simulink library "lib_TCML"  (R2015a)
settings: Solver=ode45  StartTime=0.0  StopTime=10.0  RelTol=1e-3
libraries: simulink x5
(part 1 of 7)
settings Model: Creator=jlkratz  LastModifiedBy=jlkratz

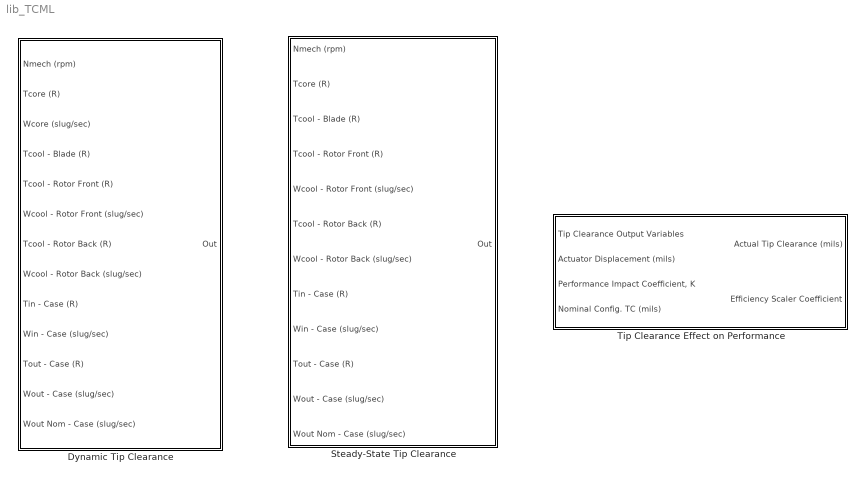
== system lib_TCML ==
  Dynamic Tip Clearance : Subsystem  mask(TCML - Dynamic Tip Clearance Library Block){m_Blade_M=0.0566, A_Blade_M=0.0174, Cp_TempDependence_Blade_M=on, Cp_Blade_M=4.5, TCp_Blade_Data_M=[0 10000], Cp_Blade_Data_M=[4.5 4.5], eta_Blade_M=0.5, T0_Blade_M=1800, dt_Blade_M=0.015, h_Const_Blade_M=off, h_Eqn_Blade_M=on, h_Data_Blade_M=off, h_Blade_M=0.03, hcoeff_Blade_M=0.03, Wdes_Blade_M=3, Tdes_Blade_M=1800, Wc_Blade_Data_M=[0 100], Tc_Blade_Data_M=[0 10], h_Blade_Data_M=[0.03 0.03; 0.03 0.03], L_Blade_M=0.125, rho_Blade_M=15.8975, alpha_TempDependence_Blade_M=on, alpha_Blade_M=0.000008, Talpha_Blade_Data_M=[0 10000], alpha_Blade_Data_M=[0.000008 0.000008], E_TempDependence_Blade_M=on, E_Blade_M=3974400000, TE_Blade_Data_M=[0 10000], E_Blade_Data_M=[3974400000 3974400000], W_Rotor_M=0.0833, n_Rotor_M=20, T0_Rotor_M=700*ones(1,20), dt_Rotor_M=0.06, rho_Rotor_M=15.8975, k_TempDependence_Rotor_M=on, k_Rotor_M=0.0015, Tk_Rotor_Data_M=[0 10000], k_Rotor_Data_M=[0.0015 0.0015], Cp_TempDependence_Rotor_M=on, Cp_Rotor_M=4.5, TCp_Rotor_Data_M=[0 10000], Cp_Rotor_Data_M=[4.5 4.5], h_Const_Rotor_Front_M=off, h_Eqn_Rotor_Front_M=on, h_Data_Rotor_Front_M=off, h_Rotor_Front_M=0.03, hcoeff_Rotor_Front_M=0.003, Wdes_Rotor_Front_M=1, Tdes_Rotor_Front_M=700, Wc_Rotor_Front_Data_M=[0 100], Tc_Rotor_Front_Data_M=[0 10], h_Rotor_Front_Data_M=[0.003 0.003; 0.003 0.003], h_Const_Rotor_Back_M=off, h_Eqn_Rotor_Back_M=on, h_Data_Rotor_Back_M=off, h_Rotor_Back_M=0.03, hcoeff_Rotor_Back_M=0.003, Wdes_Rotor_Back_M=1, Tdes_Rotor_Back_M=700, Wc_Rotor_Back_Data_M=[0 100], Tc_Rotor_Back_Data_M=[0 10], h_Rotor_Back_Data_M=[0.003 0.003; 0.003 0.003], Ro_Rotor_M=1, alpha_TempDependence_Rotor_M=on, alpha_Rotor_M=0.000008, Talpha_Rotor_Data_M=[0 10000], alpha_Rotor_Data_M=[0.000008 0.000008], E_TempDependence_Rotor_M=on, E_Rotor_M=3974400000, TE_Rotor_Data_M=[0 10000], E_Rotor_Data_M=[3974400000 3974400000], v_TempDependence_Rotor_M=on, v_Rotor_M=0.3, Tv_Rotor_Data_M=[0 10000], v_Rotor_Data_M=[0.3 0.3], W_Case_M=0.125/12, n_Case_M=20, T0_Case_M=1400*ones(1,20), dt_Case_M=0.045, rho_Case_M=15.8975, k_TempDependence_Case_M=off, k_Case_M=0.0015, Tk_Case_Data_M=[0 10000], k_Case_Data_M=[0.0015 0.0015], Cp_TempDependence_Case_M=on, Cp_Case_M=4.5, TCp_Case_Data_M=[0 10000], Cp_Case_Data_M=[4.5 4.5], h_Const_Case_In_M=off, h_Eqn_Case_In_M=on, h_Data_Case_In_M=off, h_Case_In_M=0.004, hcoeff_Case_In_M=0.04, Wdes_Case_In_M=0.03, Tdes_Case_In_M=1400, Wc_Case_In_Data_M=[0 100], Tc_Case_In_Data_M=[0 10], h_Case_In_Data_M=[0.004 0.004; 0.004 0.004], h_Const_Case_Out_M=off, h_Eqn_Case_Out_M=on, h_Data_Case_Out_M=off, h_Case_Out_M=0.004, hcoeff_Case_Out_M=0.004, Wdes_Case_Out_M=0.05, Tdes_Case_Out_M=1400, Wc_Case_Out_Data_M=[0 100], Tc_Case_Out_Data_M=[0 10], h_Case_Out_Data_M=[0.003 0.003; 0.003 0.003], Ri_Case_M=1.25, L_Shroud_M=1/12, alpha_TempDependence_Case_M=on, alpha_Case_M=0.000008, Talpha_Case_Data_M=[0 10000], alpha_Case_Data_M=[0.000008 0.000008], dt_M=0.015, T0_Core_M=2500, W0_Core_M=7, Tcool0_Blade_M=1000, Tcool0_Rotor_Front_M=700, Wcool0_Rotor_Front_M=1, Tcool0_Rotor_Back_M=700, Wcool0_Rotor_Back_M=1, Tcool0_Case_In_M=700, Wcool0_Case_In_M=1, Tcool0_Case_Out_M=700, Wcool0_Case_Out_M=1, Wcool0_Case_Out_Nom_M=0}
      mask prompts: m_Blade_M "m_Blade_M - Mass of the blade (slug) [1x1]"; A_Blade_M "A_Blade_M - Effective surface area of the blade (ft^2) [1x1]"; Cp_TempDependence_Blade_M "Cp_TempDependence_Blade_M - Heat capacity temperature dependence (unchecked - Cp = constant, checked - Cp is temperature dependent)"; Cp_Blade_M "Cp_Blade_M - Constant specific heat (Btu/(slug-R)) [1x1]"; TCp_Blade_Data_M "TCp_Blade_Data_M - Temperature data array for interpolating the heat capacity (R) [ax1]"; Cp_Blade_Data_M "Cp_Blade_Data_M - Heat capacity data array for interpolating the heat capacity (Btu/(slug-R)) [ax1]"; eta_Blade_M "eta_Blade_M - Film cooling coefficient [1x1]"; T0_Blade_M "T0_Blade_M - Initial temperature of the blade (R) [1x1]"; dt_Blade_M "dt_Blade_M - Time-step of the thermal model of the blade (sec) [1x1]"; h_Const_Blade_M "h_Const_Blade_M - Constant convective heat transfer coefficient (Btu/(sec-ft^2-R)) [1x1]"; h_Eqn_Blade_M "h_Eqn_Blade_M - h = hcoeff*(T/Tdes)^0.23*(W/Wdes)^0.8 [1x1]"; h_Data_Blade_M "h_Data_Blade_M - h = f(T/Tdes, W/Wdes) based on data [1x1]"; h_Blade_M "h_Blade_M - Constant convective heat transfer coefficient (Btu/(sec-ft^2-R)) [1x1]"; hcoeff_Blade_M "hcoeff_Blade_M - Coefficient in the convective heat transfer coefficient model h = hcoeff*(T/Tdes)^0.23*(W/Wdes)^0.8 [1x1]"; Wdes_Blade_M "Wdes_Blade_M - Design mass flow rate of core flow for a known convective heat transfer coefficient (slug/sec) [1x1]"; Tdes_Blade_M "Tdes_Blade_M - Design temperature of core flow for a known convective heat transfer coefficient (Btu/(slug-R)) [1x1]"; Wc_Blade_Data_M "Wc_Blade_Data_M - Non-dimensional mass flow rate (W/Wdes) data array for determining the convective heat transfer coefficient [bx1]"; Tc_Blade_Data_M "Tc_Blade_Data_M - Non-dimensional temperature (T/Tdes) array for determining the convective heat transfer coefficient [cx1]"; h_Blade_Data_M "h_Blade_Data_M - Matrix of convective heat transfer coefficients with rows corresponding to W/Wdes and columns corresponding to T/Tdes (Btu/(sec-ft^2-R)) [bxc]"; L_Blade_M "L_Blade_M - Blade length (ft) [1x1]"; rho_Blade_M "rho_Blade_M - Blade density (slug/ft^3) [1x1]"; alpha_TempDependence_Blade_M "alpha_TempDependence_Blade_M - Thermal expansion coefficient temperature dependence (unchecked - alpha = constant, checked - alpha is temperature dependent)"; alpha_Blade_M "alpha_Blade_M - Constant thermal expansion coefficient (1/R) [1x1]"; Talpha_Blade_Data_M "Talpha_Blade_Data_M - Temperature array for interpolating the thermal expansion coefficient (R) [dx1]"; alpha_Blade_Data_M "alpha_Blade_Data_M - Thermal expansion coefficient array for interpolating the thermal expansion coefficient (1/R) [dx1]"; E_TempDependence_Blade_M "E_TempDependence_Blade_M - Young's Modulus temperature dependence (unchecked - E = constant, checked - E is temperature dependent)"; E_Blade_M "E_Blade_M - Constant Young's Modulus (lbf/ft^2) [1x1]"; TE_Blade_Data_M "TE_Blade_Data_M - Temperature array for interpolating Young's Modulus (R) [ex1]"; E_Blade_Data_M "E_Blade_Data_M - Young's Modulus array for interpolating Young's Modulus (lbf/ft^2) [ex1]"; W_Rotor_M "W_Rotor_M - Width of the rotor (ft) [1x1]"; n_Rotor_M "n_Rotor_M - Number of nodes in spatial discretization [1x1]"; T0_Rotor_M "T0_Rotor_M - Intial temperature array (R) [n_Rotor_Mx1]"; dt_Rotor_M "dt_Rotor_M - Time-step (sec) [1x1]"; rho_Rotor_M "rho_Rotor_M - Rotor density (slug/ft^3) [1x1]"; k_TempDependence_Rotor_M "k_TempDependence_Rotor_M - Thermal conductivity temperature dependence (unchecked - k = constant, checked - k is temperature dependent)"; k_Rotor_M "k_Rotor_M - Constant thermal conductivity (Btu/(sec-ft-R)) [1x1]"; Tk_Rotor_Data_M "Tk_Rotor_Data_M - Temperature array for interpolating the thermal conductivity (R) [fx1]"; k_Rotor_Data_M "k_Rotor_Data_M - Thermal conductivity array for interpolating the thermal conductivity (Btu/(sec-ft-R)) [fx1]"; Cp_TempDependence_Rotor_M "Cp_TempDependence_Rotor_M - Heat capacity temperature dependence (unchecked - Cp = constant, checked - Cp is temperature dependent)"; Cp_Rotor_M "Cp_Rotor_M - Constant heat capacity (Btu/slug-R) [1x1]"; TCp_Rotor_Data_M "TCp_Rotor_Data_M - Temperature array for interpolating heat capacity (R) [gx1]"; Cp_Rotor_Data_M "Cp_Rotor_Data_M - Heat capacity array for interpolating heat capacity (Btu/slug-R) [gx1]"; h_Const_Rotor_Front_M "h_Const_Rotor_Front_M - Constant convective heat transfer coefficient (Btu/(sec-ft^2-R))"; h_Eqn_Rotor_Front_M "h_Eqn_Rotor_Front_M - h = hcoeff*(T/Tdes)^0.23*(W/Wdes)^0.8"; h_Data_Rotor_Front_M "h_Data_Rotor_Front_M = h = f(T/Tdes, W/Wdes) based on data"; h_Rotor_Front_M "h_Rotor_Front_M - Constant convective heat transfer coefficient (Btu/(sec-ft^2-R)) [1x1]"; hcoeff_Rotor_Front_M "hcoeff_Rotor_Front_M - Coefficient in the convective heat transfer coefficient model h = hcoeff*(T/Tdes)^0.23*(W/Wdes)^0.8 [1x1]"; Wdes_Rotor_Front_M "Wdes_Rotor_Front_M - Design mass flow rate of core flow for a known convective heat transfer coefficient (slug/sec) [1x1]"; Tdes_Rotor_Front_M "Tdes_Rotor_Front_M - Design temperature of core flow for a known convective heat transfer coefficient (Btu/(slug-R)) [1x1]"; Wc_Rotor_Front_Data_M "Wc_Rotor_Front_Data_M - Non-dimensional mass flow rate (W/Wdes) data array for determining the convective heat transfer coefficient [hx1]"; Tc_Rotor_Front_Data_M "Tc_Rotor_Front_Data_M - Non-dimensional temperature (T/Tdes) array for determining the convective heat transfer coefficient [ix1]"; h_Rotor_Front_Data_M "h_Rotor_Front_Data_M - Matrix of convective heat transfer coefficients with rows corresponding to W/Wdes and columns corresponding to T/Tdes (Btu/(sec-ft^2-R)) [hxi]"; h_Const_Rotor_Back_M "h_Const_Rotor_Back_M - Constant convective heat transfer coefficient (Btu/(sec-ft^2-R))"; h_Eqn_Rotor_Back_M "h_Eqn_Rotor_Back_M - h = hcoeff*(T/Tdes)^0.23*(W/Wdes)^0.8"; h_Data_Rotor_Back_M "h_Data_Rotor_Back_M - h = f(T/Tdes, W/Wdes) based on data"; h_Rotor_Back_M "h_Rotor_Back_M - Constant convective heat transfer coefficient (Btu/(sec-ft^2-R)) [1x1]"; hcoeff_Rotor_Back_M "hcoeff_Rotor_Back_M - Coefficient in the convective heat transfer coefficient model h = hcoeff*(T/Tdes)^0.23*(W/Wdes)^0.8 [1x1]"; Wdes_Rotor_Back_M "Wdes_Rotor_Back_M - Design mass flow rate of core flow for a known convective heat transfer coefficient (slug/sec) [1x1]"; Tdes_Rotor_Back_M "Tdes_Rotor_Back_M - Design temperature of core flow for a known convective heat transfer coefficient (Btu/(slug-R)) [1x1]"; Wc_Rotor_Back_Data_M "Wc_Rotor_Back_Data_M - Non-dimensional mass flow rate (W/Wdes) data array for determining the convective heat transfer coefficient [jx1]"; Tc_Rotor_Back_Data_M "Tc_Rotor_Back_Data_M - Non-dimensional temperature (T/Tdes) array for determining the convective heat transfer coefficient [kx1]"; h_Rotor_Back_Data_M "h_Rotor_Back_Data_M - Matrix of convective heat transfer coefficients with rows corresponding to W/Wdes and columns corresponding to T/Tdes (Btu/(sec-ft^2-R)) [jxk]"; Ro_Rotor_M "Ro_Rotor_M - Outer radius of the rotor (ft) [1x1]"; alpha_TempDependence_Rotor_M "alpha_TempDependence_Rotor_M - Thermal expansion coefficient temperature dependence (unchecked - alpha = constant, checked - alpha is temperature dependent)"; alpha_Rotor_M "alpha_Rotor_M - Constant thermal expansion coefficient (1/R) [1x1]"; Talpha_Rotor_Data_M "Talpha_Rotor_Data_M - Temperature array for interpolating the thermal expansion coefficient (R) [lx1]"; alpha_Rotor_Data_M "alpha_Rotor_Data_M - Thermal expansion coefficient array for interpolating the thermal expansion coefficient (1/R) [lx1]"; E_TempDependence_Rotor_M "E_TempDependence_Rotor_M - Young's Modulus temperature dependence (uncheck - E = constant, checked - E is temperature dependent)"; E_Rotor_M "E_Rotor_M - Constant Young's Modulus (lbf/ft^2) [1x1]"; TE_Rotor_Data_M "TE_Rotor_Data_M - Temperature array for interpolating Young's Modulus (R) [mx1]"; E_Rotor_Data_M "E_Rotor_Data_M - Young's Modulus array for interpolating Young's Modulus (lbf/ft^2) [mx1]"; v_TempDependence_Rotor_M "v_TempDependence_Rotor_M - Poisson's Ratio temperature dependence"; v_Rotor_M "v_Rotor_M - Constant Poisson's ratio [1x1]"; Tv_Rotor_Data_M "Tv_Rotor_Data_M - Temperature array for interpolating Poisson's ratio (R) [nx1]"; v_Rotor_Data_M "v_Rotor_Data_M - Poisson's ratio array for interpolating Poisson's ratio [nx1]"; W_Case_M "W_Case_M - Width of the case (ft) [1x1"; n_Case_M "n_Case_M - Number of nodes in the spatial discretization [1x1]"; T0_Case_M "T0_Case_M - Initial temperature array (R) [(n_Case_Mx1"; dt_Case_M "dt_Case_M - Time-step (sec) [1x1]"; rho_Case_M "rho_Case_M - Density (slug/ft^3) [1x1]"; k_TempDependence_Case_M "k_TempDependence_Case_M - Thermal conductivity temperature dependence (unchecked - k = constant, checked - k is temperature dependent)"; k_Case_M "k_Case_M - Constant thermal conductivity (Btu/(sec-ft-R)) [1x1]"; Tk_Case_Data_M "Tk_Case_Data_M - Temperature array for interpolating thermal conductivity (R) [qx1]"; k_Case_Data_M "k_Case_Data_M - Thermal conductivity array for interpolating thermal conductivity (Btu/(sec-ft-R)) [qx1]"; Cp_TempDependence_Case_M "Cp_TempDependence_Case_M - heat capacity temperature dependence (unchecked - Cp = constant, checked - Cp is temperature dependent)"; Cp_Case_M "Cp_Case_M - Constant heat capacity (Btu/slug-R) [1x1"; TCp_Case_Data_M "TCp_Case_Data_M - Temperature array for interpolating heat capacity (R) [rx1]"; Cp_Case_Data_M "Cp_Case_Data_M - Heat capacity array for interpolating heat capacity (Btu/slug-R) [rx1]"; h_Const_Case_In_M "h_Const_Case_In_M - Constant convective heat transfer coefficient (Btu/(sec-ft^2-R))"; h_Eqn_Case_In_M "h_Eqn_Case_In_M - h = hcoeff*(T/Tdes)^0.23*(W/Wdes)^0.8"; h_Data_Case_In_M "h_Data_Case_In_M - h = f(T/Tdes, W/Wdes) based on data"; h_Case_In_M "h_Case_In_M - Constant convective heat transfer coefficient (Btu/(sec-ft^2-R)) [1x1]"; hcoeff_Case_In_M "hcoeff_Case_In_M - Coefficient in the convective heat transfer coefficient model h = hcoeff*(T/Tdes)^0.23*(W/Wdes)^0.8 [1x1]"; Wdes_Case_In_M "Wdes_Case_In_M - Design mass flow rate of core flow for a known convective heat transfer coefficient (slug/sec) [1x1]"; Tdes_Case_In_M "Tdes_Case_In_M - Design temperature of core flow for a known convective heat transfer coefficient (Btu/(slug-R)) [1x1]"; Wc_Case_In_Data_M "Wc_Case_In_Data_M - Non-dimensional mass flow rate (W/Wdes) data array for determining the convective heat transfer coefficient [sx1]"; Tc_Case_In_Data_M "Tc_Case_In_Data_M - Non-dimensional temperature (T/Tdes) array for determining the convective heat transfer coefficient [tx1]"; h_Case_In_Data_M "h_Case_In_Data_M - Matrix of convective heat transfer coefficients with rows corresponding to W/Wdes and columns corresponding to T/Tdes (Btu/(sec-ft^2-R)) [sxt]"; h_Const_Case_Out_M "h_Const_Case_Out_M - Constant convective heat transfer coefficient (Btu/(sec-ft^2-R))"; h_Eqn_Case_Out_M "h_Eqn_Case_Out_M - h = hcoeff*(T/Tdes)^0.23*(W/Wdes)^0.8"; h_Data_Case_Out_M "h_Data_Case_Out_M - h = f(T/Tdes, W/Wdes) based on data"; h_Case_Out_M "h_Case_Out_M - Constant convective heat transfer coefficient (Btu/(sec-ft^2-R)) [1x1]"; hcoeff_Case_Out_M "hcoeff_Case_Out_M - Coefficient in the convective heat transfer coefficient model h = hcoeff*(T/Tdes)^0.23*(W/Wdes)^0.8 [1x1]"; Wdes_Case_Out_M "Wdes_Case_Out_M - Design mass flow rate of core flow for a known convective heat transfer coefficient (slug/sec) [1x1]"; Tdes_Case_Out_M "Tdes_Case_Out_M - Design temperature of core flow for a known convective heat transfer coefficient (Btu/(slug-R)) [1x1]"; Wc_Case_Out_Data_M "Wc_Case_Out_Data_M - Non-dimensional mass flow rate (W/Wdes) data array for determining the convective heat transfer coefficient [ux1]"; Tc_Case_Out_Data_M "Tc_Case_Out_Data_M - Non-dimensional temperature (T/Tdes) array for determining the convective heat transfer coefficient [vx1]"; h_Case_Out_Data_M "h_Case_Out_Data_M - Matrix of convective heat transfer coefficients with rows corresponding to W/Wdes and columns corresponding to T/Tdes (Btu/(sec-ft^2-R)) [uxv]"; Ri_Case_M "Ri_Case_M - Inner radius of the case (ft) [1x1]"; L_Shroud_M "L_Shroud_M - Distrance between the inner surface of the shroud and inner surface of the case (ft) [1x1]"; alpha_TempDependence_Case_M "alpha_TempDependence_Case_M - Thermal expansion coefficient temperature dependence (unchecked - alpha = constant, checked - alpha is temperature dependent)"; alpha_Case_M "alpha_Case_M - Constant thermal expansion coefficient (1/R) [1x1]"; Talpha_Case_Data_M "Talpha_Case_Data_M - Temperature array for interpolating the thermal expansion coefficient (R) [yx1]"; alpha_Case_Data_M "alpha_Case_Data_M - Thermal expansion coefficient array for interpolating the thermal expansion coefficient (1/R) [yx1]"; dt_M "dt_M - Time-step of the simulation outside of the tip clearance block (sec)"; T0_Core_M "T0_Core_M - Initial temperature of the core flow (R)"; W0_Core_M "W0_Core_M - Initial mass flow rate of the core flow (slug/sec)"; Tcool0_Blade_M "Tcool0_Blade_M - Intial temperature of the cooling air for the blade  (R)"; Tcool0_Rotor_Front_M "Tcool0_Rotor_Front_M - Initial temperature of the cooling air for the front of the rotor (R)"; Wcool0_Rotor_Front_M "Wcool0_Rotor_Front_M - Initial mass flow rate of the cooling air for the front of the rotor (slug/sec)"; Tcool0_Rotor_Back_M "Tcool0_Rotor_Back_M - Initial temperature of the cooling air for the back of the rotor (R)"; Wcool0_Rotor_Back_M "Wcool0_Rotor_Back_M  - Initial mass flow rate of the cooling air for the back of the rotor (slug/sec)"; Tcool0_Case_In_M "Tcool0_Case_In_M - Initial  temperature of cooling air on the inner surface of the case (R)"; Wcool0_Case_In_M "Wcool0_Case_In_M - Initial mass flow rate of cooling air on the inner surface of the case (slug/sec)"; Tcool0_Case_Out_M "Tcool0_Case_Out_M - Initial  temperature of cooling air on the outer surface of the case (R)"; Wcool0_Case_Out_M "Wcool0_Case_Out_M - Initial mass flow rate of cooling air on the outer surface of the case (slug/sec)"; Wcool0_Case_Out_Nom_M "Wcool0_Case_Out_Nom_M - Initial nominal flow rate on the outer case [slug/sec]"
      mask help:
      | This block is identical to the 'Tip Clearance' library block with the exception that it will eliminate and add inports as they are applicable to the settings specified in the parameter dialog box. If the input is unnecessary for the given setting then it will be removed.
      |
      | This function approximates axisymmetric tip clearance variation inside turbomachinery (i.e. compressors and turbines). It models the deformation of the rotor, blade, and case/shroud (containment structure) due to elastic thermal and centrifugal deformation. The blade is modeled as a lumped mass and the rotor and case use a 1-D finite difference approach for temperature determination. The deformation of the shroud is assumed to be governed by the deformation of the case that supports it. The thermal deformation models uses the average component temperature. This function has numerous options for modeling convective heat transfer coefficients and temperature dependence of various parameters including thermal conductivity, heat capacity, thermal expansion coefficient, Young's Modulus, and Poisson's ratio.
      |
      | Units of the inputs and parameters are indicated so be sure to abide by them. See the block help menu for more details.
      mask init:
      | % check for warning/errors -----------------------------------------------%
      | 
      | % Blade -----------------------------%
      | 
      | % m_Blade_M
      | if length(m_Blade_M) ~= 1
      |     fprintf('warning in %s: m_Blade_M must be a scalar entry.\n',gcb)
      | end
      | if m_Blade_M <= 0 || isreal(m_Blade_M) == 0
      |     fprintf('warning in %s: m_Blade_M must be a real positive number.\n',gcb)
      | end
      | 
      | % A_Blade_M
      | if length(A_Blade_M) ~= 1
      |     fprintf('warning in %s: A_Blade_M must be a scalar entry.\n',gcb)
      | end
      | if A_Blade_M <= 0 || isreal(A_Blade_M) == 0
      |     fprintf('warning in %s: A_Blade_M must be a real positive number.\n',gcb)
      | end
      | 
      | % Cp_Blade_M
      | if length(Cp_Blade_M) ~= 1
      |     fprintf('warning in %s: Cp_Blade_M must be a scalar entry.\n',gcb)
      | end
      | if Cp_Blade_M <= 0 || isreal(Cp_Blade_M) == 0
      |     fprintf('warning in %s: Cp_Blade_M must be a real positive number.\n',gcb)
      | end
      | 
      | % TCp_Blade_Data_M & Cp_Blade_Data_M
      | if length(TCp_Blade_Data_M) < 2
      |     fprintf('warning in %s: TCp_Blade_Data_M must have at least 2 elements.\n',gcb)
      | end
      | if length(Cp_Blade_Data_M) < 2
      |     fprintf('warning in %s: Cp_Blade_Data_M must have at least 2 elements.\n',gcb)
      | end
      | if length(TCp_Blade_Data_M) ~= length(Cp_Blade_Data_M)
      |     fprintf('warning in %s: TCp_Blade_Data_M and Cp_Blade_Data_M must have the same dimensions.\n',gcb)
      | end
      | real_TCp_Blade_Data_M = isreal(TCp_Blade_Data_M);
      | if min(real_TCp_Blade_Data_M) == 0
      |     fprintf('warning in %s: TCp_Blade_Data_M must have all real entries.\n',gcb)
      | end
      | diff_TCp_Blade_Data_M = diff(TCp_Blade_Data_M);
      | if min(diff_TCp_Blade_Data_M) <= 0
      |     fprintf('warning in %s: TCp_Blade_Data_M must be monotonically increasing.\n',gcb)
      | end
      | if min(TCp_Blade_Data_M) < 0
      |     fprintf('warning in %s: Elements of TCp_Blade_Data_M are below 0 which is theoretically impossible.\n',gcb)
      | end
      | real_Cp_Blade_Data_M = isreal(Cp_Blade_Data_M);
      | if min(real_Cp_Blade_Data_M) == 0
      |     fprintf('warning in %s: Cp_Blade_Data_M must have all real entries.\n',gcb)
      | end
      | if min(Cp_Blade_Data_M) <= 0
      |     fprintf('warning in %s: Elements of Cp_Blade_Data_M are below 0 which is impossible.\n',gcb)
      | end
      | 
      | % eta_Blade_M
      | if length(eta_Blade_M) ~= 1
      |     fprintf('warning in %s: eta_Blade_M must be a scalar entry.\n',gcb)
      | end
      | if eta_Blade_M < 0 || eta_Blade_M > 1
      |     fprintf('warning in %s: eta_Blade_M must be between 0 and 1.\n',gcb)
      | end
      | 
      | % T0_Blade_M
      | if length(T0_Blade_M) ~= 1
      |     fprintf('warning in %s: T0_Blade_M must be a scalar entry.\n',gcb)
      | end
      | if T0_Blade_M < 0 || isreal(T0_Blade_M) == 0
      |     fprintf('warning in %s: T0_Blade_M must be a real positive number.\n',gcb)
      | end
      | 
      | % dt_Blade_M
      | if dt_Blade_M < 0 || isreal(dt_Blade_M) == 0
      |     fprintf('warning in %s: dt_Blade_M must be a real positive number.\n',gcb)
      | end
      | 
      | % h_Blade_M
      | if length(h_Blade_M) ~= 1
      |     fprintf('warning in %s: h_Blade_M must be a scalar.\n',gcb)
      | end
      | if h_Blade_M < 0 || isreal(h_Blade_M) == 0
      |     fprintf('warning in %s: h_Blade_M must be a real positive entry.\n',gcb)
      | end
      | 
      | % hcoeff_Blade_M
      | if length(hcoeff_Blade_M) ~= 1
      |     fprintf('warning in %s: hcoeff_Blade_M must be a scalar.\n',gcb)
      | end
      | if hcoeff_Blade_M < 0 || isreal(hcoeff_Blade_M) == 0
      |     fprintf('warning in %s: hcoeff_Blade_M must be a real positive entry.\n',gcb)
      | end
      | 
      | % Wdes_Blade_M
      | if length(Wdes_Blade_M) ~= 1
      |     fprintf('warning in %s: Wdes_Blade_M must be a scalar entry.\n',gcb)
      | end
      | if Wdes_Blade_M <= 0 || isreal(Wdes_Blade_M) == 0
      |     fprintf('warning in %s: Wdes_Blade_M must be a real positive number.\n',gcb)
      | end
      | 
      | % Tdes_Blade_M
      | if length(Tdes_Blade_M) ~= 1
      |     fprintf('warning in %s: Tdes_Blade_M must be a scalar entry.\n',gcb)
      | end
      | if Tdes_Blade_M <= 0 || isreal(Tdes_Blade_M) == 0
      |     fprintf('warning in %s: Tdes_Blade_M must be a real positive number.\n',gcb)
      | end
      | 
      | % Wc_Blade_Data_M, Tc_Blade_Data_M & h_Blade_Data_M
      | [nR, nC] = size(h_Blade_Data_M);
      | if nR < 2 || nC < 2
      |     fprintf('warning in %s: h_Blade_Data_M must be a matrix of at least 2 rows and 2 columns.\n',gcb)
      | end
      | if length(Wc_Blade_Data_M) ~= nR
      |     fprintf('warning in %s: Wc_Blade_Data_M must have the same number of elements as rows in h_Blade_Data_M.\n',gcb)
      | end
      | if length(Tc_Blade_Data_M) ~= nC
      |     fprintf('warning in %s: Tc_Blade_Data_M must have the same number of elements as columns in h_Blade_Data_M.\n',gcb)
      | end
      | real_Wc_Blade_Data_M = isreal(Wc_Blade_Data_M);
      | if min(real_Wc_Blade_Data_M) == 0
      |     fprintf('warning in %s: Wc_Blade_Data_M must have all real entries.\n',gcb)
      | end
      | diff_Wc_Blade_Data_M = diff(Wc_Blade_Data_M);
      | if min(diff_Wc_Blade_Data_M) <= 0
      |     fprintf('warning in %s: Wc_Blade_Data_M must be monotonically increasing.\n',gcb)
      | end
      | real_Tc_Blade_Data_M = isreal(Tc_Blade_Data_M);
      | if min(real_Tc_Blade_Data_M) == 0
      |     fprintf('warning in %s: Tc_Blade_Data_M must have all real entries.\n',gcb)
      | end
      | diff_Tc_Blade_Data_M = diff(Tc_Blade_Data_M);
      | if min(diff_Tc_Blade_Data_M) <= 0
      |     fprintf('warning in %s: Tc_Blade_Data_M must be monotonically increasing.\n',gcb)
      | end
      | if min(Tc_Blade_Data_M) < 0
      |     fprintf('warning in %s: Elements of Tc_Blade_Data_M are less than 0 which is impossible.\n',gcb)
      | end
      | real_h_Blade_Data_M = isreal(h_Blade_Data_M);
      | if min(real_h_Blade_Data_M) == 0 || min(min(h_Blade_Data_M)) < 0
      |     fprintf('warning in %s: h_Blade_Data_M must have all real positive entries.\n',gcb)
      | end
      | 
      | % L_Blade_M
      | if length(L_Blade_M) ~= 1
      |     fprintf('warning in %s: L_Blade_M must be a scalar entry.\n',gcb)
      | end
      | if L_Blade_M <= 0 || isreal(L_Blade_M) == 0
      |     fprintf('warning in %s: L_Blade_M must be a real positive number.\n',gcb)
      | end
      | 
      | % rho_Blade_M
      | if length(rho_Blade_M) ~= 1
      |     fprintf('warning in %s: rho_Blade_M must be a scalar entry.\n',gcb)
      | end
      | if rho_Blade_M <= 0 || isreal(rho_Blade_M) == 0
      |     fprintf('warning in %s: rho_Blade_M must be a real positive number.\n',gcb)
      | end
      | 
      | % E_Blade_M
      | if length(E_Blade_M) ~= 1
      |     fprintf('warning in %s: E_Blade_M must be a scalar entry.\n',gcb)
      | end
      | if E_Blade_M <= 0 || isreal(E_Blade_M) == 0
      |     fprintf('warning in %s: E_Blade_M must be a real positive number.\n',gcb)
      | end
      | 
      | % TE_Blade_Data_M & E_Blade_Data_M
      | if length(TE_Blade_Data_M) < 2
      |     fprintf('warning in %s: TE_Blade_Data_M must have at least 2 elements.\n',gcb)
      | end
      | if length(E_Blade_Data_M) < 2
      |     fprintf('warning in %s: E_Blade_Data_M must have at least 2 elements.\n',gcb)
      | end
      | if length(TE_Blade_Data_M) ~= length(E_Blade_Data_M)
      |     fprintf('warning in %s: TE_Blade_Data_M and E_Blade_Data_M must have the same dimensions.\n',gcb)
      | end
      | real_TE_Blade_Data_M = isreal(TE_Blade_Data_M);
      | if min(real_TE_Blade_Data_M) == 0
      |     fprintf('warning in %s: TE_Blade_Data_M must have all real entries.\n',gcb)
      | end
      | diff_TE_Blade_Data_M = diff(TE_Blade_Data_M);
      | if min(diff_TE_Blade_Data_M) <= 0
      |     fprintf('warning in %s: TE_Blade_Data_M must be monotonically increasing.\n',gcb)
      | end
      | if min(TE_Blade_Data_M) < 0
      |     fprintf('warning in %s: Elements of TE_Blade_Data_M are below 0 which is theoretically impossible.\n',gcb)
      | end
      | real_E_Blade_Data_M = isreal(E_Blade_Data_M);
      | if min(real_E_Blade_Data_M) == 0
      |     fprintf('warning in %s: E_Blade_Data_M must have all real entries.\n',gcb)
      | end
      | if min(E_Blade_Data_M) <= 0
      |     fprintf('warning in %s: Elements of E_Blade_Data_M are below 0 which is impossible.\n',gcb)
      | end
      | 
      | % Blade variables checked by underlying blocks:
      | %   alpha_Blade_M
      | %   Talpha_Blade_Data_M
      | %   alpha_Blade_Data_M
      | 
      | % Rotor --------------------------%
      | 
      | % W_Rotor_M
      | if length(W_Rotor_M) ~= 1
      |     fprintf('warning in %s: W_Rotor_M must be a scalar entry.\n',gcb)
      | end
      | if W_Rotor_M <= 0 || isreal(W_Rotor_M) == 0
      |     fprintf('warning in %s: W_Rotor_M must be a real positive number.\n',gcb)
      | end
      | 
      | % n_Rotor_M
      | if length(n_Rotor_M) ~= 1
      |     fprintf('warning in %s: n_Rotor_M must be a scalar entry.\n',gcb)
      | end
      | if n_Rotor_M <= 0 || isreal(n_Rotor_M) == 0
      |     fprintf('warning in %s: n_Rotor_M must be a real positive number.\n',gcb)
      | end
      | if n_Rotor_M < 4
      |     fprintf('warning in %s: n_Rotor_M must be >= 4.\n',gcb)
      | end
      | 
      | % rho_Rotor_M
      | if length(rho_Rotor_M) ~= 1
      |     fprintf('warning in %s: rho_Rotor_M must be a scalar entry.\n',gcb)
      | end
      | if rho_Rotor_M <= 0 || isreal(rho_Rotor_M) == 0
      |     fprintf('warning in %s: rho_Rotor_M must be a real positive number.\n',gcb)
      | end
      | 
      | % k_Rotor_M
      | if length(k_Rotor_M) ~= 1
      |     fprintf('warning in %s: k_Rotor_M must be a scalar entry.\n',gcb)
      | end
      | if k_Rotor_M <= 0 || isreal(k_Rotor_M) == 0
      |     fprintf('warning in %s: k_Rotor_M must be a real positive number.\n',gcb)
      | end
      | 
      | % Tk_Rotor_Data_M & k_Rotor_Data_M
      | if length(Tk_Rotor_Data_M) < 2
      |     fprintf('warning in %s: Tk_Rotor_Data_M must have at least 2 elements.\n',gcb)
      | end
      | if length(k_Rotor_Data_M) < 2
      |     fprintf('warning in %s: k_Rotor_Data_M must have at least 2 elements.\n',gcb)
      | end
      | if length(Tk_Rotor_Data_M) ~= length(k_Rotor_Data_M)
      |     fprintf('warning in %s: Tk_Rotor_Data_M and k_Rotor_Data_M must have the same dimensions.\n',gcb)
      | end
      | real_Tk_Rotor_Data_M = isreal(Tk_Rotor_Data_M);
      | if min(real_Tk_Rotor_Data_M) == 0
      |     fprintf('warning in %s: Tk_Rotor_Data_M must have all real entries.\n',gcb)
      | end
      | diff_Tk_Rotor_Data_M = diff(Tk_Rotor_Data_M);
      | if min(diff_Tk_Rotor_Data_M) <= 0
      |     fprintf('warning in %s: Tk_Rotor_Data_M must be monotonically increasing.\n',gcb)
      | end
      | if min(Tk_Rotor_Data_M) < 0
      |     fprintf('warning in %s: Elements of Tk_Rotor_Data_M are below 0 which is theoretically impossible.\n',gcb)
      | end
      | real_k_Rotor_Data_M = isreal(k_Rotor_Data_M);
      | if min(real_k_Rotor_Data_M) == 0
      |     fprintf('warning in %s: k_Rotor_Data_M must have all real entries.\n',gcb)
      | end
      | if min(k_Rotor_Data_M) <= 0
      |     fprintf('warning in %s: Elements of k_Rotor_Data_M are below 0 which is impossible.\n',gcb)
      | end
      | 
      | % Cp_Rotor_M
      | if length(Cp_Rotor_M) ~= 1
      |     fprintf('warning in %s: Cp_Rotor_M must be a scalar entry.\n',gcb)
      | end
      | if Cp_Rotor_M <= 0 || isreal(Cp_Rotor_M) == 0
      |     fprintf('warning in %s: Cp_Rotor_M must be a real positive number.\n',gcb)
      | end
      | 
      | % TCp_Rotor_Data_M & Cp_Rotor_Data_M
      | if length(TCp_Rotor_Data_M) < 2
      |     fprintf('warning in %s: TCp_Rotor_Data_M must have at least 2 elements.\n',gcb)
      | end
      | if length(Cp_Rotor_Data_M) < 2
      |     fprintf('warning in %s: Cp_Rotor_Data_M must have at least 2 elements.\n',gcb)
      | end
      | if length(TCp_Rotor_Data_M) ~= length(Cp_Rotor_Data_M)
      |     fprintf('warning in %s: TCp_Rotor_Data_M and Cp_Rotor_Data_M must have the same dimensions.\n',gcb)
      | end
      | real_TCp_Rotor_Data_M = isreal(TCp_Rotor_Data_M);
      | if min(real_TCp_Rotor_Data_M) == 0
      |     fprintf('warning in %s: TCp_Rotor_Data_M must have all real entries.\n',gcb)
      | end
      | diff_TCp_Rotor_Data_M = diff(TCp_Rotor_Data_M);
      | if min(diff_TCp_Rotor_Data_M) <= 0
      |     fprintf('warning in %s: TCp_Rotor_Data_M must be monotonically increasing.\n',gcb)
      | end
      | if min(TCp_Rotor_Data_M) < 0
      |     fprintf('warning in %s: Elements of TCp_Rotor_Data_M are below 0 which is theoretically impossible.\n',gcb)
      | end
      | real_Cp_Rotor_Data_M = isreal(Cp_Rotor_Data_M);
      | if min(real_Cp_Rotor_Data_M) == 0
      |     fprintf('warning in %s: Cp_Rotor_Data_M must have all real entries.\n',gcb)
      | end
      | if min(Cp_Rotor_Data_M) <= 0
      |     fprintf('warning in %s: Elements of Cp_Rotor_Data_M are below 0 which is impossible.\n',gcb)
      | end
      | 
      | % hcoeff_Rotor_Front_M
      | if length(hcoeff_Rotor_Front_M) ~= 1
      |     fprintf('warning in %s: hcoeff_Rotor_Front_M must be a scalar.\n',gcb)
      | end
      | if hcoeff_Rotor_Front_M < 0 || isreal(hcoeff_Rotor_Front_M) == 0
      |     fprintf('warning in %s: hcoeff_Rotor_Front_M must be a real positive entry.\n',gcb)
      | end
      | 
      | % Wdes_Rotor_Front_M
      | if length(Wdes_Rotor_Front_M) ~= 1
      |     fprintf('warning in %s: Wdes_Rotor_Front_M must be a scalar entry.\n',gcb)
      | end
      | if Wdes_Rotor_Front_M <= 0 || isreal(Wdes_Rotor_Front_M) == 0
      |     fprintf('warning in %s: Wdes_Rotor_Front_M must be a real positive number.\n',gcb)
      | end
      | 
      | % Tdes_Rotor_Front_M
      | if length(Tdes_Rotor_Front_M) ~= 1
      |     fprintf('warning in %s: Tdes_Rotor_Front_M must be a scalar entry.\n',gcb)
      | end
      | if Tdes_Rotor_Front_M <= 0 || isreal(Tdes_Rotor_Front_M) == 0
      |     fprintf('warning in %s: Tdes_Rotor_Front_M must be a real positive number.\n',gcb)
      | end
      | 
      | % Wc_Rotor_Front_Data_M, Tc_Rotor_Front_Data_M & h_Rotor_Front_Data_M
      | [nR, nC] = size(h_Rotor_Front_Data_M);
      | if nR < 2 || nC < 2
      |     fprintf('warning in %s: h_Rotor_Front_Data_M must be a matrix of at least 2 rows and 2 columns.\n',gcb)
      | end
      | if length(Wc_Rotor_Front_Data_M) ~= nR
      |     fprintf('warning in %s: Wc_Rotor_Front_Data_M must have the same number of elements as rows in h_Rotor_Front_Data_M.\n',gcb)
      | end
      | if length(Tc_Rotor_Front_Data_M) ~= nC
      |     fprintf('warning in %s: Tc_Rotor_Front_Data_M must have the same number of elements as columns in h_Rotor_Front_Data_M.\n',gcb)
      | end
      | real_Wc_Rotor_Front_Data_M = isreal(Wc_Rotor_Front_Data_M);
      | if min(real_Wc_Blade_Data_M) == 0
      |     fprintf('warning in %s: Wc_Rotor_Front_Data_M must have all real entries.\n',gcb)
      | end
      | diff_Wc_Rotor_Front_Data_M = diff(Wc_Rotor_Front_Data_M);
      | if min(diff_Wc_Rotor_Front_Data_M) <= 0
      |     fprintf('warning in %s: Wc_Rotor_Front_Data_M must be monotonically increasing.\n',gcb)
      | end
      | real_Tc_Rotor_Front_Data_M = isreal(Tc_Rotor_Front_Data_M);
      | if min(real_Tc_Rotor_Front_Data_M) == 0
      |     fprintf('warning in %s: Tc_Rotor_Front_Data_M must have all real entries.\n',gcb)
      | end
      | diff_Tc_Rotor_Front_Data_M = diff(Tc_Rotor_Front_Data_M);
      | if min(diff_Tc_Rotor_Front_Data_M) <= 0
      |     fprintf('warning in %s: Tc_Rotor_Front_Data_M must be monotonically increasing.\n',gcb)
      | end
      | if min(Tc_Blade_Data_M) < 0
      |     fprintf('warning in %s: Elements of Tc_Rotor_Front_Data_M are less than 0 which is impossible.\n',gcb)
      | end
      | real_h_Rotor_Front_Data_M = isreal(h_Rotor_Front_Data_M);
      | if min(real_h_Rotor_Front_Data_M) == 0 || min(min(h_Rotor_Front_Data_M)) < 0
      |     fprintf('warning in %s: h_Rotor_Front_Data_M must have all real positive entries.\n',gcb)
      | end
      | 
      | % hcoeff_Rotor_Back_M
      | if length(hcoeff_Rotor_Back_M) ~= 1
      |     fprintf('warning in %s: hcoeff_Rotor_Back_M must be a scalar.\n',gcb)
      | end
      | if hcoeff_Rotor_Back_M < 0 || isreal(hcoeff_Rotor_Back_M) == 0
      |     fprintf('warning in %s: hcoeff_Rotor_Back_M must be a real positive entry.\n',gcb)
      | end
      | 
      | % Wdes_Rotor_Back_M
      | if length(Wdes_Rotor_Back_M) ~= 1
      |     fprintf('warning in %s: Wdes_Rotor_Back_M must be a scalar entry.\n',gcb)
      | end
      | if Wdes_Rotor_Back_M <= 0 || isreal(Wdes_Rotor_Back_M) == 0
      |     fprintf('warning in %s: Wdes_Rotor_Back_M must be a real positive number.\n',gcb)
      | end
      | 
      | % Tdes_Rotor_Back_M
      | if length(Tdes_Rotor_Back_M) ~= 1
      |     fprintf('warning in %s: Tdes_Rotor_Back_M must be a scalar entry.\n',gcb)
      | end
      | if Tdes_Rotor_Back_M <= 0 || isreal(Tdes_Rotor_Back_M) == 0
      |     fprintf('warning in %s: Tdes_Rotor_Back_M must be a real positive number.\n',gcb)
      | end
      | 
      | % Wc_Rotor_Back_Data_M, Tc_Rotor_Back_Data_M & h_Rotor_Back_Data_M
      | [nR, nC] = size(h_Rotor_Back_Data_M);
      | if nR < 2 || nC < 2
      |     fprintf('warning in %s: h_Rotor_Back_Data_M must be a matrix of at least 2 rows and 2 columns.\n',gcb)
      | end
      | if length(Wc_Rotor_Back_Data_M) ~= nR
      |     fprintf('warning in %s: Wc_Rotor_Back_Data_M must have the same number of elements as rows in h_Rotor_Back_Data_M.\n',gcb)
      | end
      | if length(Tc_Rotor_Back_Data_M) ~= nC
      |     fprintf('warning in %s: Tc_Rotor_Back_Data_M must have the same number of elements as columns in h_Rotor_Back_Data_M.\n',gcb)
      | end
      | real_Wc_Rotor_Back_Data_M = isreal(Wc_Rotor_Back_Data_M);
      | if min(real_Wc_Rotor_Back_Data_M) == 0
      |     fprintf('warning in %s: Wc_Rotor_Back_Data_M must have all real entries.\n',gcb)
      | end
      | diff_Wc_Rotor_Back_Data_M = diff(Wc_Rotor_Back_Data_M);
      | if min(diff_Wc_Rotor_Back_Data_M) <= 0
      |     fprintf('warning in %s: Wc_Rotor_Front_Data_M must be monotonically increasing.\n',gcb)
      | end
      | real_Tc_Rotor_Back_Data_M = isreal(Tc_Rotor_Back_Data_M);
      | if min(real_Tc_Rotor_Back_Data_M) == 0
      |     fprintf('warning in %s: Tc_Rotor_Back_Data_M must have all real entries.\n',gcb)
      | end
      | diff_Tc_Rotor_Back_Data_M = diff(Tc_Rotor_Back_Data_M);
      | if min(diff_Tc_Rotor_Back_Data_M) <= 0
      |     fprintf('warning in %s: Tc_Rotor_Back_Data_M must be monotonically increasing.\n',gcb)
      | end
      | if min(Tc_Rotor_Back_Data_M) < 0
      |     fprintf('warning in %s: Elements of Tc_Rotor_Back_Data_M are less than 0 which is impossible.\n',gcb)
      | end
      | real_h_Rotor_Back_Data_M = isreal(h_Rotor_Back_Data_M);
      | if min(real_h_Rotor_Back_Data_M) == 0 || min(min(h_Rotor_Back_Data_M)) < 0
      |     fprintf('warning in %s: h_Rotor_Back_Data_M must have all real positive entries.\n',gcb)
      | end
      | 
      | % Ro_Rotor_M
      | if length(Ro_Rotor_M) ~= 1
      |     fprintf('warning in %s: Ro_Rotor_M must be a scalar entry.\n',gcb)
      | end
      | if Ro_Rotor_M <= 0 || isreal(Ro_Rotor_M) == 0
      |     fprintf('warning in %s: Ro_Rotor_M must be a real positive number.\n',gcb)
      | end
      | 
      | % E_Rotor_M
      | if length(E_Rotor_M) ~= 1
      |     fprintf('warning in %s: E_Rotor_M must be a scalar entry.\n',gcb)
      | end
      | if E_Rotor_M <= 0 || isreal(E_Rotor_M) == 0
      |     fprintf('warning in %s: E_Rotor_M must be a real positive number.\n',gcb)
      | end
      | 
      | % TE_Rotor_Data_M & E_Rotor_Data_M
      | if length(TE_Rotor_Data_M) < 2
      |     fprintf('warning in %s: TE_Rotor_Data_M must have at least 2 elements.\n',gcb)
      | end
      | if length(E_Rotor_Data_M) < 2
      |     fprintf('warning in %s: E_Rotor_Data_M must have at least 2 elements.\n',gcb)
      | end
      | if length(TE_Rotor_Data_M) ~= length(E_Rotor_Data_M)
      |     fprintf('warning in %s: TE_Rotor_Data_M and E_Rotor_Data_M must have the same dimensions.\n',gcb)
      | end
      | real_TE_Rotor_Data_M = isreal(TE_Rotor_Data_M);
      | if min(real_TE_Rotor_Data_M) == 0
      |     fprintf('warning in %s: TE_Rotor_Data_M must have all real entries.\n',gcb)
      | end
      | diff_TE_Rotor_Data_M = diff(TE_Rotor_Data_M);
      | if min(diff_TE_Rotor_Data_M) <= 0
      |     fprintf('warning in %s: TE_Rotor_Data_M must be monotonically increasing.\n',gcb)
      | end
      | if min(TE_Rotor_Data_M) < 0
      |     fprintf('warning in %s: Elements of TE_Rotor_Data_M are below 0 which is theoretically impossible.\n',gcb)
      | end
      | real_E_Rotor_Data_M = isreal(E_Rotor_Data_M);
      | if min(real_E_Rotor_Data_M) == 0
      |     fprintf('warning in %s: E_Rotor_Data_M must have all real entries.\n',gcb)
      | end
      | if min(E_Rotor_Data_M) <= 0
      |     fprintf('warning in %s: Elements of E_Rotor_Data_M are below 0 which is impossible.\n',gcb)
      | end
      | 
      | % v_Rotor_M
      | if length(v_Rotor_M) ~= 1
      |     fprintf('warning in %s: v_Rotor_M must be a scalar entry.\n',gcb)
      | end
      | if isreal(v_Rotor_M) == 0
      |     fprintf('warning in %s: E_Rotor_M must be a real number.\n',gcb)
      | end
      | 
      | % Tv_Rotor_Data_M & v_Rotor_Data_M
      | if length(Tv_Rotor_Data_M) < 2
      |     fprintf('warning in %s: Tv_Rotor_Data_M must have at least 2 elements.\n',gcb)
      | end
      | if length(v_Rotor_Data_M) < 2
      |     fprintf('warning in %s: v_Rotor_Data_M must have at least 2 elements.\n',gcb)
      | end
      | if length(Tv_Rotor_Data_M) ~= length(v_Rotor_Data_M)
      |     fprintf('warning in %s: Tv_Rotor_Data_M and v_Rotor_Data_M must have the same dimensions.\n',gcb)
      | end
      | real_Tv_Rotor_Data_M = isreal(Tv_Rotor_Data_M);
      | if min(real_Tv_Rotor_Data_M) == 0
      |     fprintf('warning in %s: Tv_Rotor_Data_M must have all real entries.\n',gcb)
      | end
      | diff_Tv_Rotor_Data_M = diff(Tv_Rotor_Data_M);
      | if min(diff_Tv_Rotor_Data_M) <= 0
      |     fprintf('warning in %s: Tv_Rotor_Data_M must be monotonically increasing.\n',gcb)
      | end
      | if min(Tv_Rotor_Data_M) < 0
      |     fprintf('warning in %s: Elements of Tv_Rotor_Data_M are below 0 which is theoretically impossible.\n',gcb)
      | end
      | real_E_Rotor_Data_M = isreal(v_Rotor_Data_M);
      | if min(real_E_Rotor_Data_M) == 0
      |     fprintf('warning in %s: v_Rotor_Data_M must have all real entries.\n',gcb)
      | end
      | 
      | % Rotor variables checked by underlying blocks:
      | %   T0_Rotor_M
      | %   dt_Rotor_M
      | %   alpha_Rotor_M
      | %   Talpah_Rotor_Data_M
      | %   alpha_Rotor_Data_M
      | 
      | % Case --------------------------%
      | 
      | % W_Case_M
      | if length(W_Case_M) ~= 1
      |     fprintf('warning in %s: W_Case_M must be a scalar entry.\n',gcb)
      | end
      | if W_Case_M <= 0 || isreal(W_Case_M) == 0
      |     fprintf('warning in %s: W_Case_M must be a real positive number.\n',gcb)
      | end
      | 
      | % n_Case_M
      | if length(n_Case_M) ~= 1
      |     fprintf('warning in %s: n_Case_M must be a scalar entry.\n',gcb)
      | end
      | if n_Case_M <= 0 || isreal(n_Case_M) == 0
      |     fprintf('warning in %s: n_Case_M must be a real positive number.\n',gcb)
      | end
      | if n_Case_M < 4
      |     fprintf('warning in %s: n_Case_M must be >= 4.\n',gcb)
      | end
      | 
      | % rho_Case_M
      | if length(rho_Case_M) ~= 1
      |     fprintf('warning in %s: rho_Case_M must be a scalar entry.\n',gcb)
      | end
      | if rho_Case_M <= 0 || isreal(rho_Case_M) == 0
      |     fprintf('warning in %s: rho_Case_M must be a real positive number.\n',gcb)
      | end
      | 
      | % k_Case_M
      | if length(k_Case_M) ~= 1
      |     fprintf('warning in %s: k_Case_M must be a scalar entry.\n',gcb)
      | end
      | if k_Case_M <= 0 || isreal(k_Case_M) == 0
      |     fprintf('warning in %s: k_Case_M must be a real positive number.\n',gcb)
      | end
      | 
      | % Tk_Case_Data_M & k_Case_Data_M
      | if length(Tk_Case_Data_M) < 2
      |     fprintf('warning in %s: Tk_Case_Data_M must have at least 2 elements.\n',gcb)
      | end
      | if length(k_Case_Data_M) < 2
      |     fprintf('warning in %s: k_Case_Data_M must have at least 2 elements.\n',gcb)
      | end
      | if length(Tk_Case_Data_M) ~= length(k_Case_Data_M)
      |     fprintf('warning in %s: Tk_Case_Data_M and k_Case_Data_M must have the same dimensions.\n',gcb)
      | end
      | real_Tk_Case_Data_M = isreal(Tk_Case_Data_M);
      | if min(real_Tk_Case_Data_M) == 0
      |     fprintf('warning in %s: Tk_Case_Data_M must have all real entries.\n',gcb)
      | end
      | diff_Tk_Case_Data_M = diff(Tk_Case_Data_M);
      | if min(diff_Tk_Case_Data_M) <= 0
      |     fprintf('warning in %s: Tk_Case_Data_M must be monotonically increasing.\n',gcb)
      | end
      | if min(Tk_Case_Data_M) < 0
      |     fprintf('warning in %s: Elements of Tk_Case_Data_M are below 0 which is theoretically impossible.\n',gcb)
      | end
      | real_k_Case_Data_M = isreal(k_Case_Data_M);
      | if min(real_k_Case_Data_M) == 0
      |     fprintf('warning in %s: k_Case_Data_M must have all real entries.\n',gcb)
      | end
      | if min(k_Case_Data_M) <= 0
      |     fprintf('warning in %s: Elements of k_Case_Data_M are below 0 which is impossible.\n',gcb)
      | end
      | 
      | % Cp_Case_M
      | if length(Cp_Case_M) ~= 1
      |     fprintf('warning in %s: Cp_Case_M must be a scalar entry.\n',gcb)
      | end
      | if Cp_Case_M <= 0 || isreal(Cp_Case_M) == 0
      |     fprintf('warning in %s: Cp_Case_M must be a real positive number.\n',gcb)
      | end
      | 
      | % TCp_Case_Data_M & Cp_Case_Data_M
      | if length(TCp_Case_Data_M) < 2
      |     fprintf('warning in %s: TCp_Case_Data_M must have at least 2 elements.\n',gcb)
      | end
      | if length(Cp_Case_Data_M) < 2
      |     fprintf('warning in %s: Cp_Case_Data_M must have at least 2 elements.\n',gcb)
      | end
      | if length(TCp_Case_Data_M) ~= length(Cp_Case_Data_M)
      |     fprintf('warning in %s: TCp_Case_Data_M and Cp_Case_Data_M must have the same dimensions.\n',gcb)
      | end
      | real_TCp_Case_Data_M = isreal(TCp_Case_Data_M);
      | if min(real_TCp_Case_Data_M) == 0
      |     fprintf('warning in %s: TCp_Case_Data_M must have all real entries.\n',gcb)
      | end
      | diff_TCp_Case_Data_M = diff(TCp_Case_Data_M);
      | if min(diff_TCp_Case_Data_M) <= 0
      |     fprintf('warning in %s: TCp_Case_Data_M must be monotonically increasing.\n',gcb)
      | end
      | if min(TCp_Case_Data_M) < 0
      |     fprintf('warning in %s: Elements of TCp_Case_Data_M are below 0 which is theoretically impossible.\n',gcb)
      | end
      | real_Cp_Case_Data_M = isreal(Cp_Case_Data_M);
      | if min(real_Cp_Case_Data_M) == 0
      |     fprintf('warning in %s: Cp_Case_Data_M must have all real entries.\n',gcb)
      | end
      | if min(Cp_Case_Data_M) <= 0
      |     fprintf('warning in %s: Elements of Cp_Case_Data_M are below 0 which is impossible.\n',gcb)
      | end
      | 
      | % hcoeff_Case_In_M
      | if length(hcoeff_Case_In_M) ~= 1
      |     fprintf('warning in %s: hcoeff_Case_In_M must be a scalar.\n',gcb)
      | end
      | if hcoeff_Case_In_M < 0 || isreal(hcoeff_Case_In_M) == 0
      |     fprintf('warning in %s: hcoeff_Case_In_M must be a real positive entry.\n',gcb)
      | end
      | 
      | % Wdes_Case_In_M
      | if length(Wdes_Case_In_M) ~= 1
      |     fprintf('warning in %s: Wdes_Case_In_M must be a scalar entry.\n',gcb)
      | end
      | if Wdes_Case_In_M <= 0 || isreal(Wdes_Case_In_M) == 0
      |     fprintf('warning in %s: Wdes_Case_In_M must be a real positive number.\n',gcb)
      | end
      | 
      | % Tdes_Case_In_M
      | if length(Tdes_Case_In_M) ~= 1
      |     fprintf('warning in %s: Tdes_Case_In_M must be a scalar entry.\n',gcb)
      | end
      | if Tdes_Case_In_M <= 0 || isreal(Tdes_Case_In_M) == 0
      |     fprintf('warning in %s: Tdes_Case_In_M must be a real positive number.\n',gcb)
      | end
      | 
      | % Wc_Case_In_Data_M, Tc_Case_In_Data_M & h_Case_In_Data_M
      | [nR, nC] = size(h_Case_In_Data_M);
      | if nR < 2 || nC < 2
      |     fprintf('warning in %s: h_Case_In_Data_M must be a matrix of at least 2 rows and 2 columns.\n',gcb)
      | end
      | if length(Wc_Case_In_Data_M) ~= nR
      |     fprintf('warning in %s: Wc_Case_In_Data_M must have the same number of elements as rows in h_Case_In_Data_M.\n',gcb)
      | end
      | if length(Tc_Case_In_Data_M) ~= nC
      |     fprintf('warning in %s: Tc_Case_In_Data_M must have the same number of elements as columns in h_Case_In_Data_M.\n',gcb)
      | end
      | real_Wc_Case_In_Data_M = isreal(Wc_Case_In_Data_M);
      | if min(real_Wc_Case_In_Data_M) == 0
      |     fprintf('warning in %s: Wc_Case_In_Data_M must have all real entries.\n',gcb)
      | end
      | diff_Wc_Case_In_Data_M = diff(Wc_Case_In_Data_M);
      | if min(diff_Wc_Case_In_Data_M) <= 0
      |     fprintf('warning in %s: Wc_Case_In_Data_M must be monotonically increasing.\n',gcb)
      | end
      | real_Tc_Case_In_Data_M = isreal(Tc_Case_In_Data_M);
      | if min(real_Tc_Case_In_Data_M) == 0
      |     fprintf('warning in %s: Tc_Case_In_Data_M must have all real entries.\n',gcb)
      | end
      | diff_Tc_Case_In_Data_M = diff(Tc_Case_In_Data_M);
      | if min(diff_Tc_Case_In_Data_M) <= 0
      |     fprintf('warning in %s: Tc_Case_In_Data_M must be monotonically increasing.\n',gcb)
      | end
      | if min(Tc_Case_In_Data_M) < 0
      |     fprintf('warning in %s: Elements of Tc_Case_In_Data_M are less than 0 which is impossible.\n',gcb)
      | end
      | real_h_Case_In_Data_M = isreal(h_Case_In_Data_M);
      | if min(real_h_Case_In_Data_M) == 0 || min(min(h_Case_In_Data_M)) < 0
      |     fprintf('warning in %s: h_Case_In_Data_M must have all real positive entries.\n',gcb)
      | end
      | 
      | % hcoeff_Case_Out_M
      | if length(hcoeff_Case_Out_M) ~= 1
      |     fprintf('warning in %s: hcoeff_Case_Out_M must be a scalar.\n',gcb)
      | end
      | if hcoeff_Case_Out_M < 0 || isreal(hcoeff_Case_Out_M) == 0
      |     fprintf('warning in %s: hcoeff_Case_Out_M must be a real positive entry.\n',gcb)
      | end
      | 
      | % Wdes_Case_Out_M
      | if length(Wdes_Case_Out_M) ~= 1
      |     fprintf('warning in %s: Wdes_Case_Out_M must be a scalar entry.\n',gcb)
      | end
      | if Wdes_Case_Out_M <= 0 || isreal(Wdes_Case_Out_M) == 0
      |     fprintf('warning in %s: Wdes_Case_Out_M must be a real positive number.\n',gcb)
      | end
      | 
      | % Tdes_Case_Out_M
      | if length(Tdes_Case_Out_M) ~= 1
      |     fprintf('warning in %s: Tdes_Case_Out_M must be a scalar entry.\n',gcb)
      | end
      | if Tdes_Case_Out_M <= 0 || isreal(Tdes_Case_Out_M) == 0
      |     fprintf('warning in %s: Tdes_Case_Out_M must be a real positive number.\n',gcb)
      | end
      | 
      | % Wc_Case_Out_Data_M, Tc_Case_Out_Data_M & h_Case_Out_Data_M
      | [nR, nC] = size(h_Case_Out_Data_M);
      | if nR < 2 || nC < 2
      |     fprintf('warning in %s: h_Case_Out_Data_M must be a matrix of at least 2 rows and 2 columns.\n',gcb)
      | end
      | if length(Wc_Case_Out_Data_M) ~= nR
      |     fprintf('warning in %s: Wc_Case_Out_Data_M must have the same number of elements as rows in h_Case_Out_Data_M.\n',gcb)
      | end
      | if length(Tc_Case_Out_Data_M) ~= nC
      |     fprintf('warning in %s: Tc_Case_Out_Data_M must have the same number of elements as columns in h_Case_Out_Data_M.\n',gcb)
      | end
      | real_Wc_Case_Out_Data_M = isreal(Wc_Case_Out_Data_M);
      | if min(real_Wc_Case_Out_Data_M) == 0
      |     fprintf('warning in %s: Wc_Case_Out_Data_M must have all real entries.\n',gcb)
      | end
      | diff_Wc_Case_Out_Data_M = diff(Wc_Case_Out_Data_M);
      | if min(diff_Wc_Case_Out_Data_M) <= 0
      |     fprintf('warning in %s: Wc_Case_Out_Data_M must be monotonically increasing.\n',gcb)
      | end
      | real_Tc_Case_Out_Data_M = isreal(Tc_Case_Out_Data_M);
      | if min(real_Tc_Case_Out_Data_M) == 0
      |     fprintf('warning in %s: Tc_Case_Out_Data_M must have all real entries.\n',gcb)
      | end
      | diff_Tc_Case_Out_Data_M = diff(Tc_Case_Out_Data_M);
      | if min(diff_Tc_Case_Out_Data_M) <= 0
      |     fprintf('warning in %s: Tc_Case_Out_Data_M must be monotonically increasing.\n',gcb)
      | end
      | if min(Tc_Case_Out_Data_M) < 0
      |     fprintf('warning in %s: Elements of Tc_Case_Out_Data_M are less than 0 which is impossible.\n',gcb)
      | end
      | real_h_Case_Out_Data_M = isreal(h_Case_Out_Data_M);
      | if min(real_h_Case_Out_Data_M) == 0 || min(min(h_Case_Out_Data_M)) < 0
      |     fprintf('warning in %s: h_Case_Out_Data_M must have all real positive entries.\n',gcb)
      | end
      | 
      | % Ri_Case_M
      | if length(Ri_Case_M) ~= 1
      |     fprintf('warning in %s: Ri_Case_M must be a scalar entry.\n',gcb)
      | end
      | if Ri_Case_M <= 0 || isreal(Ri_Case_M) == 0
      |     fprintf('warning in %s: Ri_Case_M must be a real positive number.\n',gcb)
      | end
      | 
      | % L_Shroud_M
      | if length(L_Shroud_M) ~= 1
      |     fprintf('warning in %s: L_Shroud_M must be a scalar entry.\n',gcb)
      | end
      | if L_Shroud_M <= 0 || isreal(L_Shroud_M) == 0
      |     fprintf('warning in %s: L_Shroud_M must be a real positive number.\n',gcb)
      | end
      | 
      | % Case variables checked by underlying blocks:
      | %   T0_Case_M
      | %   dt_Case_M
      | %   alpha_Case_M
      | %   Talpha_Case_Data_M
      | %   alpha_Case_data_M
      | 
      | % BC initialization -----------------%
      | 
      | % T0_Core_M
      | if length(T0_Core_M) ~= 1
      |     fprintf('warning in %s: T0_Core_M must be a scalar entry.\n',gcb)
      | end
      | if T0_Core_M <= 0 || isreal(T0_Core_M) == 0
      |     fprintf('warning in %s: T0_Core_M must be a real positive number.\n',gcb)
      | end
      | 
      | % W0_Core_M
      | if length(W0_Core_M) ~= 1
      |     fprintf('warning in %s: W0_Core_M must be a scalar entry.\n',gcb)
      | end
      | if isreal(W0_Core_M) == 0
      |     fprintf('warning in %s: W0_Core_M must be a real number.\n',gcb)
      | end
      | 
      | % Tcool0_Blade_M
      | if length(Tcool0_Blade_M) ~= 1
      |     fprintf('warning in %s: Tcool0_Blade_M must be a scalar entry.\n',gcb)
      | end
      | if Tcool0_Blade_M <= 0 || isreal(Tcool0_Blade_M) == 0
      |     fprintf('warning in %s: Tcool0_Blade_M must be a real positive number.\n',gcb)
      | end
      | 
      | % Tcool0_Rotor_Front_M
      | if length(Tcool0_Rotor_Front_M) ~= 1
      |     fprintf('warning in %s: Tcool0_Rotor_Front_M must be a scalar entry.\n',gcb)
      | end
      | if Tcool0_Rotor_Front_M <= 0 || isreal(Tcool0_Rotor_Front_M) == 0
      |     fprintf('warning in %s: Tcool0_Rotor_Front_M must be a real positive number.\n',gcb)
      | end
      | 
      | % Wcool0_Rotor_Front_M
      | if length(Wcool0_Rotor_Front_M) ~= 1
      |     fprintf('warning in %s: Wcool0_Rotor_Front_M must be a scalar entry.\n',gcb)
      | end
      | if isreal(Wcool0_Rotor_Front_M) == 0
      |     fprintf('warning in %s: Wcool0_Rotor_Front_M must be a real number.\n',gcb)
      | end
      | 
      | % Tcool0_Rotor_Back_M
      | if length(Tcool0_Rotor_Back_M) ~= 1
      |     fprintf('warning in %s: Tcool0_Rotor_Back_M must be a scalar entry.\n',gcb)
      | end
      | if Tcool0_Rotor_Back_M <= 0 || isreal(Tcool0_Rotor_Back_M) == 0
      |     fprintf('warning in %s: Tcool0_Rotor_Back_M must be a real positive number.\n',gcb)
      | end
      | 
      | % Wcool0_Rotor_Back_M
      | if length(Wcool0_Rotor_Back_M) ~= 1
      |     fprintf('warning in %s: Wcool0_Rotor_Back_M must be a scalar entry.\n',gcb)
      | end
      | if isreal(Wcool0_Rotor_Back_M) == 0
      |     fprintf('warning in %s: Wcool0_Rotor_Back_M must be a real number.\n',gcb)
      | end
      | 
      | % Tcool0_Case_In_M
      | if length(Tcool0_Case_In_M) ~= 1
      |     fprintf('warning in %s: Tcool0_Case_In_M must be a scalar entry.\n',gcb)
      | end
      | if Tcool0_Case_In_M <= 0 || isreal(Tcool0_Case_In_M) == 0
      |     fprintf('warning in %s: Tcool0_Case_In_M must be a real positive number.\n',gcb)
      | end
      | 
      | % Wcool0_Case_In_M
      | if length(Wcool0_Case_In_M) ~= 1
      |     fprintf('warning in %s: Wcool0_Case_In_M must be a scalar entry.\n',gcb)
      | end
      | if isreal(Wcool0_Case_In_M) == 0
      |     fprintf('warning in %s: Wcool0_Case_In_M must be a real number.\n',gcb)
      | end
      | 
      | % Tcool0_Case_Out_M
      | if length(Tcool0_Case_Out_M) ~= 1
      |     fprintf('warning in %s: Tcool0_Case_Out_M must be a scalar entry.\n',gcb)
      | end
      | if Tcool0_Case_Out_M <= 0 || isreal(Tcool0_Case_Out_M) == 0
      |     fprintf('warning in %s: Tcool0_Case_Out_M must be a real positive number.\n',gcb)
      | end
      | 
      | % Wcool0_Case_Out_M
      | if length(Wcool0_Case_Out_M) ~= 1
      |     fprintf('warning in %s: Wcool0_Case_Out_M must be a scalar entry.\n',gcb)
      | end
      | if isreal(Wcool0_Case_Out_M) == 0
      |     fprintf('warning in %s: Wcool0_Case_Out_M must be a real number.\n',gcb)
      | end
      | 
      | % time-step agreement ---------------%
      | dt_min = min([dt_Blade_M dt_Rotor_M dt_Case_M dt_M]);
      | if rem(dt_Blade_M,dt_min) ~= 0 
      |     fprintf('warning in %s: dt_Blade_M must be a multiple of the minimum time-step in the simulation. Changing value to the closest non-zero multiple.\n',gcb)
      |     dt_Blade = round(dt_Blade_M/dt_min)*dt_min;
      |     if dt_Blade_M == 0
      |         dt_Blade_M = dt_min;
      |     end
      | end
      | if rem(dt_Rotor_M,dt_min) ~= 0 
      |     fprintf('warning in %s: dt_Rotor_M must be a multiple of the minimum time-step in the simulation. Changing value to the closest non-zero multiple.\n',gcb)
      |     dt_Rotor_M = round(dt_Rotor_M/dt_min)*dt_min;
      |     if dt_Rotor_M == 0
      |         dt_Rotor_M = dt_min;
      |     end
      | end
      | if rem(dt_Case_M,dt_min) ~= 0 
      |     fprintf('warning in %s: dt_Case_M must be a multiple of the minimum time-step in the simulation. Changing value to the closest non-zero multiple.\n',gcb)
      |     dt_Case_M = round(dt_Case_M/dt_min)*dt_min;
      |     if dt_Case_M == 0
      |         dt_Case_M = dt_min;
      |     end
      | end
      | if rem(dt_M,dt_min) ~= 0 
      |     fprintf('warning in %s: dt_M must be a multiple of the minimum time-step in the simulation. Changing value to the closest non-zero multiple.\n',gcb)
      |     dt_M = round(dt_M/dt_min)*dt_min;
      |     if dt_M == 0
      |         dt_M = dt_min;
      |     end
      | end
      | 
      | % calculate intialization parameters -------------------------------------%
      | 
      | % Rotor discretization (node locations)
      | dx_Rotor = W_Rotor_M/(n_Rotor_M-1); %node thickness
      | x_Rotor_I = [0:dx_Rotor:W_Rotor_M]; %discretization array [ft]
      | 
      | % Case discretization (nodel locations)
      | dx_Case = W_Case_M/(n_Case_M-1); %node thickness
      | x_Case_I = Ri_Case_M + [0:dx_Case:W_Case_M]; %discretizaiton array [ft]
      | 
      | % Convection Model selection variables
      | % Blade
      | if h_Const_Blade_M == 1
      |     ConvHeatXCoeffMdl_Blade_I = 1;
      | elseif h_Eqn_Blade_M == 1
      |     ConvHeatXCoeffMdl_Blade_I = 2;
      | elseif h_Data_Blade_M == 1
      |     ConvHeatXCoeffMdl_Blade_I = 3;
      | end
      | % Rotor-Front
      | if h_Const_Rotor_Front_M == 1
      |     ConvHeatXCoeffMdl_Rotor_Front_I = 1;
      | elseif h_Eqn_Rotor_Front_M == 1
      |     ConvHeatXCoeffMdl_Rotor_Front_I = 2;
      | elseif h_Data_Rotor_Front_M == 1
      |     ConvHeatXCoeffMdl_Rotor_Front_I = 3;
      | end
      | % Rotor-Back
      | if h_Const_Rotor_Back_M == 1
      |     ConvHeatXCoeffMdl_Rotor_Back_I = 1;
      | elseif h_Eqn_Rotor_Back_M == 1
      |     ConvHeatXCoeffMdl_Rotor_Back_I = 2;
      | elseif h_Data_Rotor_Back_M == 1
      |     ConvHeatXCoeffMdl_Rotor_Back_I = 3;
      | end
      | % Case-In
      | if h_Const_Case_In_M == 1
      |     ConvHeatXCoeffMdl_Case_In_I = 1;
      | elseif h_Eqn_Case_In_M == 1
      |     ConvHeatXCoeffMdl_Case_In_I = 2;
      | elseif h_Data_Case_In_M == 1
      |     ConvHeatXCoeffMdl_Case_In_I = 3;
      | end
      | % Case-Out
      | if h_Const_Case_Out_M == 1
      |     ConvHeatXCoeffMdl_Case_Out_I = 1;
      | elseif h_Eqn_Case_Out_M == 1
      |     ConvHeatXCoeffMdl_Case_Out_I = 2;
      | elseif h_Data_Case_Out_M == 1
      |     ConvHeatXCoeffMdl_Case_Out_I = 3;
      | end
      | 
      | % set thermal expansion temperature dependence settings ------------------%
      | 
      | % Blade
      | set_param([gcb,'/Blade Deformation/Deformation/Deformation Due To Thermal Expansion/Thermal Expansion 1D Elastic'],'TempDependence_M',alpha_TempDependence_Blade_M);
      |     
      | % Rotor
      | set_param([gcb,'/Rotor Deformation/Deformation/Deformation Due To Thermal Expansion/Thermal Expansion 1D Elastic'],'TempDependence_M',alpha_TempDependence_Rotor_M);
      | 
      | % Case
      | set_param([gcb,'/Case Deformation/Deformation/Thermal Expansion 1D Elastic'],'TempDependence_M',alpha_TempDependence_Case_M);
      | 
      | % set default parameters if they are not being used ----------------------%
      | 
      | % Blade
      | if Cp_TempDependence_Blade_M == 0
      |     TCp_Blade_Data_M = [0 10000];
      |     Cp_Blade_Data_M = [7.75 7.75];
      | elseif Cp_TempDependence_Blade_M == 1
      |     Cp_Blade_M = 7.75;
      | end
      | 
      | if h_Const_Blade_M == 1
      |     hcoeff_Blade_M = 0.003;
      |     Wdes_Blade_M = 1;
      |     Tdes_Blade_M = 1;
      |     Wc_Blade_Data_M = [0 10000];
      |     Tc_Blade_Data_M = [0 10000];
      |     h_Blade_Data_M = [0.003 0.003; 0.003 0.003];
      | elseif h_Eqn_Blade_M == 1
      |     h_Blade_M = 0.003;
      |     Wc_Blade_Data_M = [0 10000];
      |     Tc_Blade_Data_M = [0 10000];
      |     h_Blade_Data_M = [0.003 0.003; 0.003 0.003];
      | elseif h_Data_Blade_M == 1
      |     h_Blade_M = 0.003;
      |     hcoeff_Blade_M = 0.003;
      | end
      | 
      | if alpha_TempDependence_Blade_M == 0
      |     Talpha_Blade_Data_M = [0 10000];
      |     alpha_Blade_Data_M = [0.000001 0.000001];
      | elseif alpha_TempDependence_Blade_M == 1
      |     alpha_Blade_M = 0.000001;
      | end
      | 
      | if E_TempDependence_Blade_M == 0
      |     TE_Blade_Data_M = [0 10000];
      |     E_Blade_Data_M = [3974400000 3974400000];
      | elseif E_TempDependence_Blade_M == 1
      |     E_Blade_M = 3974400000;
      | end
      | 
      | % Rotor
      | if k_TempDependence_Rotor_M == 0
      |     Tk_Rotor_Data_M = [0 10000];
      |     k_Rotor_Data_M = [0.0015 0.0015];
      | elseif k_TempDependence_Rotor_M == 1
      |     k_Rotor_M = 0.0015;
      | end
      | 
      | if Cp_TempDependence_Rotor_M == 0
      |     TCp_Rotor_Data_M = [0 10000];
      |     Cp_Rotor_Data_M = [7.75 7.75];
      | elseif Cp_TempDependence_Rotor_M == 1
      |     Cp_Rotor_M = 7.75;
      | end
      | 
      | if h_Const_Rotor_Front_M == 1
      |     hcoeff_Rotor_Front_M = 0.003;
      |     Wdes_Rotor_Front_M = 1;
      |     Tdes_Rotor_Front_M = 1;
      |     Wc_Rotor_Front_Data_M = [0 10000];
      |     Tc_Rotor_Front_Data_M = [0 10000];
      |     h_Rotor_Front_Data_M = [0.003 0.003; 0.003 0.003];
      | elseif h_Eqn_Rotor_Front_M == 1
      |     h_Rotor_Front_M = 0.003;
      |     Wc_Rotor_Front_Data_M = [0 10000];
      |     Tc_Rotor_Front_Data_M = [0 10000];
      |     h_Rotor_Front_Data_M = [0.003 0.003; 0.003 0.003];
      | elseif h_Data_Rotor_Front_M == 1
      |     h_Rotor_Front_M = 0.003;
      |     hcoeff_Rotor_Front_M = 0.003;
      | end
      | 
      | if h_Const_Rotor_Back_M == 1
      |     hcoeff_Rotor_Back_M = 0.003;
      |     Wdes_Rotor_Back_M = 1;
      |     Tdes_Rotor_Back_M = 1;
      |     Wc_Rotor_Back_Data_M = [0 10000];
      |     Tc_Rotor_Back_Data_M = [0 10000];
      |     h_Rotor_Back_Data_M = [0.003 0.003; 0.003 0.003];
      | elseif h_Eqn_Rotor_Back_M == 1
      |     h_Rotor_Back_M = 0.003;
      |     Wc_Rotor_Back_Data_M = [0 10000];
      |     Tc_Rotor_Back_Data_M = [0 10000];
      |     h_Rotor_Back_Data_M = [0.003 0.003; 0.003 0.003];
      | elseif h_Data_Rotor_Back_M == 1
      |     h_Rotor_Back_M = 0.003;
      |     hcoeff_Rotor_Back_M = 0.003;
      | end
      | 
      | if alpha_TempDependence_Rotor_M == 0
      |     Talpha_Rotor_Data_M = [0 10000];
      |     alpha_Rotor_Data_M = [0.000001 0.000001];
      | elseif alpha_TempDependence_Rotor_M == 1
      |     alpha_Rotor_M = 0.000001;
      | end
      | 
      | if E_TempDependence_Rotor_M == 0
      |     TE_Rotor_Data_M = [0 10000];
      |     E_Rotor_Data_M = [3974400000 3974400000];
      | elseif E_TempDependence_Rotor_M == 1
      |     E_Rotor_M = 3974400000;
      | end
      | 
      | if v_TempDependence_Rotor_M == 0
      |     Tv_Rotor_Data_M = [0 10000];
      |     v_Rotor_Data_M = [0.3 0.3];
      | elseif v_TempDependence_Rotor_M == 1
      |     v_Rotor_M = 0.3;
      | end
      | 
      | % Case
      | if k_TempDependence_Case_M == 0
      |     Tk_Case_Data_M = [0 10000];
      |     k_Case_Data_M = [0.0015 0.0015];
      | elseif k_TempDependence_Case_M == 1
      |     k_Case_M = 0.0015;
      | end
      | 
      | if Cp_TempDependence_Case_M == 0
      |     TCp_Case_Data_M = [0 10000];
      |     Cp_Case_Data_M = [7.75 7.75];
      | elseif Cp_TempDependence_Case_M == 1
      |     Cp_Case_M = 7.75;
      | end
      | 
      | if h_Const_Case_In_M == 1
      |     hcoeff_Case_In_M = 0.003;
      |     Wdes_Case_In_M = 1;
      |     Tdes_Case_In_M = 1;
      |     Wc_Case_In_Data_M = [0 10000];
      |     Tc_Case_In_Data_M = [0 10000];
      |     h_Case_In_Data_M = [0.003 0.003; 0.003 0.003];
      | elseif h_Eqn_Case_In_M == 1
      |     h_Case_In_M = 0.003;
      |     Wc_Case_In_Data_M = [0 10000];
      |     Tc_Case_In_Data_M = [0 10000];
      |     h_Case_In_Data_M = [0.003 0.003; 0.003 0.003];
      | elseif h_Data_Case_In_M == 1
      |     h_Case_In_M = 0.003;
      |     hcoeff_Case_In_M = 0.003;
      | end
      | 
      | if h_Const_Case_Out_M == 1
      |     hcoeff_Case_Out_M = 0.003;
      |     Wdes_Case_Out_M = 1;
      |     Tdes_Case_Out_M = 1;
      |     Wc_Case_Out_Data_M = [0 10000];
      |     Tc_Case_Out_Data_M = [0 10000];
      |     h_Case_Out_Data_M = [0.003 0.003; 0.003 0.003];
      | elseif h_Eqn_Case_Out_M == 1
      |     h_Case_Out_M = 0.003;
      |     Wc_Case_Out_Data_M = [0 10000];
      |     Tc_Case_Out_Data_M = [0 10000];
      |     h_Case_Out_Data_M = [0.003 0.003; 0.003 0.003];
      | elseif h_Data_Case_Out_M == 1
      |     h_Case_Out_M = 0.003;
      |     hcoeff_Case_Out_M = 0.003;
      | end
      | 
      | if alpha_TempDependence_Case_M == 0
      |     Talpha_Case_Data_M = [0 10000];
      |     alpha_Case_Data_M = [0.000001 0.000001];
      | elseif alpha_TempDependence_Case_M == 1
      |     alpha_Case_M = 0.000001;
      | end
      | 
      | %BC initialization
      | if h_Const_Blade_M == 1
      |     W0_Core_M = 7;
      | end
      | 
      | if h_Const_Rotor_Front_M == 1
      |     Wcool0_Rotor_Front_M = 1;
      | end
      | 
      | if h_Const_Rotor_Back_M == 1
      |     Wcool0_Rotor_Back_M = 1;
      | end
      | 
      | if h_Const_Case_Out_M == 1
      |     Wcool0_Case_M = 3;
      | end
      | 
      | % inport and constant block swapping -------------------------------------%
      | 
      | % Inport Numbers
      | n = 3; %first inport number
      | 
      | % Core Mass Flow Rate Inport
      | if h_Const_Blade_M == 0
      |     if strcmp(get_param([gcb '/Wcore (slug//sec)'],'BlockType'),'Constant')
      |         MSK_ReplaceBlock_TMATS([gcb '/Wcore (slug//sec)'],'built-in/Inport');
      |     end
      |     set_param([gcb '/Wcore (slug//sec)'],'Port',num2str(n));
      |     n = n + 1;
      | else
      |     if strcmp(get_param([gcb '/Wcore (slug//sec)'],'BlockType'),'Inport')
      |         MSK_ReplaceBlock_TMATS([gcb '/Wcore (slug//sec)'],'built-in/Constant');
      |         set_param([gcb '/Wcore (slug//sec)'],'Value','1');
      |     end
      | end
      | 
      | % Rotor Cooling Flow Mass Flow Rate - Front Inport
      | n = n + 2;
      | if h_Const_Rotor_Front_M == 0
      |     if strcmp(get_param([gcb '/Wcool - Rotor Front (slug//sec)'],'BlockType'),'Constant')
      |         MSK_ReplaceBlock_TMATS([gcb '/Wcool - Rotor Front (slug//sec)'],'built-in/Inport');
      |     end
      |     set_param([gcb '/Wcool - Rotor Front (slug//sec)'],'Port',num2str(n));
      |     n = n + 1;
      | else
      |     if strcmp(get_param([gcb '/Wcool - Rotor Front (slug//sec)'],'BlockType'),'Inport')
      |         MSK_ReplaceBlock_TMATS([gcb '/Wcool - Rotor Front (slug//sec)'],'built-in/Constant');
      |         set_param([gcb '/Wcool - Rotor Front (slug//sec)'],'Value','1');
      |     end
      | end
      | 
      | % Rotor Cooling Flow Mass Flow Rate - Back Inport
      | n = n + 1;
      | if h_Const_Rotor_Back_M == 0
      |     if strcmp(get_param([gcb '/Wcool - Rotor Back (slug//sec)'],'BlockType'),'Constant')
      |         MSK_ReplaceBlock_TMATS([gcb '/Wcool - Rotor Back (slug//sec)'],'built-in/Inport');
      |     end
      |     set_param([gcb '/Wcool - Rotor Back (slug//sec)'],'Port',num2str(n));
      |     n = n + 1;
      | else
      |     if strcmp(get_param([gcb '/Wcool - Rotor Back (slug//sec)'],'BlockType'),'Inport')
      |         MSK_ReplaceBlock_TMATS([gcb '/Wcool - Rotor Back (slug//sec)'],'built-in/Constant');
      |         set_param([gcb '/Wcool - Rotor Back (slug//sec)'],'Value','1');
      |     end
      | end
      | 
      | % Case Cooling Flow Mass Flow Rate - Inner Inport
      | n = n + 1;
      | if h_Const_Case_In_M == 0
      |     if strcmp(get_param([gcb '/Win - Case (slug//sec)'],'BlockType'),'Constant')
      |         MSK_ReplaceBlock_TMATS([gcb '/Win - Case (slug//sec)'],'built-in/Inport');
      |     end
      |     set_param([gcb '/Win - Case (slug//sec)'],'Port',num2str(n));
      |     n = n + 1;
      | else
      |     if strcmp(get_param([gcb '/Win - Case (slug//sec)'],'BlockType'),'Inport')
      |         MSK_ReplaceBlock_TMATS([gcb '/Win - Case (slug//sec)'],'built-in/Constant');
      |         set_param([gcb '/Win - Case (slug//sec)'],'Value','1');
      |     end
      | end
      | 
      | % Case Cooling Flow Mass Flow Rate - Outer Inport
      | n = n + 1;
      | if h_Const_Case_Out_M == 0
      |     if strcmp(get_param([gcb '/Wout - Case (slug//sec)'],'BlockType'),'Constant')
      |         MSK_ReplaceBlock_TMATS([gcb '/Wout - Case (slug//sec)'],'built-in/Inport');
      |     end
      |     set_param([gcb '/Wout - Case (slug//sec)'],'Port',num2str(n));
      |     n = n + 1;
      | else
      |     if strcmp(get_param([gcb '/Wout - Case (slug//sec)'],'BlockType'),'Inport')
      |         MSK_ReplaceBlock_TMATS([gcb '/Wout - Case (slug//sec)'],'built-in/Constant');
      |         set_param([gcb '/Wout - Case (slug//sec)'],'Value','1');
      |     end
      | end
      mask Help: web(which('DynTipClearance.html'),'-helpbrowser')
      mask Callback Cp_TempDependence_Blade_M:
      | MSK_SEC_Enables_TMATS('Cp_TempDependence_Blade_M',4,'dis')
      | MSK_SEC_Enables_TMATS('Cp_TempDependence_Blade_M',[5 6],'en')
      mask Callback h_Const_Blade_M:
      | if length(get_param(gcb,'h_Const_Blade_M')) == 2 %on
      |     set_param(gcb,'h_Eqn_Blade_M','off');
      |     set_param(gcb,'h_Data_Blade_M','off');
      |     MSK_SEC_Enables2_TMATS('h_Const_Blade_M',13,'en')
      |     MSK_SEC_Enables2_TMATS('h_Const_Blade_M',[14 15 16 17 18 19 117],'dis')
      | end
      mask Callback h_Eqn_Blade_M:
      | if length(get_param(gcb,'h_Eqn_Blade_M')) == 2 %on
      |     set_param(gcb,'h_Const_Blade_M','off');
      |     set_param(gcb,'h_Data_Blade_M','off');
      |     MSK_SEC_Enables2_TMATS('h_Eqn_Blade_M',[14 15 16 117],'en')
      |     MSK_SEC_Enables2_TMATS('h_Eqn_Blade_M',[13 17 18 19],'dis')
      | end
      mask Callback h_Data_Blade_M:
      | if length(get_param(gcb,'h_Data_Blade_M')) == 2 %on
      |     set_param(gcb,'h_Eqn_Blade_M','off');
      |     set_param(gcb,'h_Const_Blade_M','off');
      |     MSK_SEC_Enables2_TMATS('h_Data_Blade_M',[13 14],'dis')
      |     MSK_SEC_Enables2_TMATS('h_Data_Blade_M',[15 16 17 18 19 117],'en')
      | end
      mask Callback alpha_TempDependence_Blade_M:
      | MSK_SEC_Enables_TMATS('alpha_TempDependence_Blade_M',23,'dis')
      | MSK_SEC_Enables_TMATS('alpha_TempDependence_Blade_M',[24 25],'en')
      mask Callback E_TempDependence_Blade_M:
      | MSK_SEC_Enables_TMATS('E_TempDependence_Blade_M',27,'dis')
      | MSK_SEC_Enables_TMATS('E_TempDependence_Blade_M',[28 29],'en')
      mask Callback k_TempDependence_Rotor_M:
      | MSK_SEC_Enables_TMATS('k_TempDependence_Rotor_M',36,'dis')
      | MSK_SEC_Enables_TMATS('k_TempDependence_Rotor_M',[37 38],'en')
      mask Callback Cp_TempDependence_Rotor_M:
      | MSK_SEC_Enables_TMATS('Cp_TempDependence_Rotor_M',40,'dis')
      | MSK_SEC_Enables_TMATS('Cp_TempDependence_Rotor_M',[41 42],'en')
      mask Callback h_Const_Rotor_Front_M:
      | if length(get_param(gcb,'h_Const_Rotor_Front_M')) == 2 %on
      |     set_param(gcb,'h_Eqn_Rotor_Front_M','off');
      |     set_param(gcb,'h_Data_Rotor_Front_M','off');
      |     MSK_SEC_Enables2_TMATS('h_Const_Rotor_Front_M',46,'en')
      |     MSK_SEC_Enables2_TMATS('h_Const_Rotor_Front_M',[47 48 49 50 51 52 120],'dis')
      | end
      mask Callback h_Eqn_Rotor_Front_M:
      | if length(get_param(gcb,'h_Eqn_Rotor_Front_M')) == 2 %on
      |     set_param(gcb,'h_Const_Rotor_Front_M','off');
      |     set_param(gcb,'h_Data_Rotor_Front_M','off');
      |     MSK_SEC_Enables2_TMATS('h_Eqn_Rotor_Front_M',[47 48 49 120],'en')
      |     MSK_SEC_Enables2_TMATS('h_Eqn_Rotor_Front_M',[46 50 51 52],'dis')
      | end
      mask Callback h_Data_Rotor_Front_M:
      | if length(get_param(gcb,'h_Data_Rotor_Front_M')) == 2 %on
      |     set_param(gcb,'h_Eqn_Rotor_Front_M','off');
      |     set_param(gcb,'h_Const_Rotor_Front_M','off');
      |     MSK_SEC_Enables2_TMATS('h_Data_Rotor_Front_M',[46 47],'dis')
      |     MSK_SEC_Enables2_TMATS('h_Data_Rotor_Front_M',[48 49 50 51 52 120],'en')
      | end
      mask Callback h_Const_Rotor_Back_M:
      | if length(get_param(gcb,'h_Const_Rotor_Back_M')) == 2 %on
      |     set_param(gcb,'h_Eqn_Rotor_Back_M','off');
      |     set_param(gcb,'h_Data_Rotor_Back_M','off');
      |     MSK_SEC_Enables2_TMATS('h_Const_Rotor_Back_M',56,'en')
      |     MSK_SEC_Enables2_TMATS('h_Const_Rotor_Back_M',[57 58 59 60 61 62 122],'dis')
      | end
      mask Callback h_Eqn_Rotor_Back_M:
      | if length(get_param(gcb,'h_Eqn_Rotor_Back_M')) == 2 %on
      |     set_param(gcb,'h_Const_Rotor_Back_M','off');
      |     set_param(gcb,'h_Data_Rotor_Back_M','off');
      |     MSK_SEC_Enables2_TMATS('h_Eqn_Rotor_Back_M',[57 58 59 122],'en')
      |     MSK_SEC_Enables2_TMATS('h_Eqn_Rotor_Back_M',[56 60 61 62],'dis')
      | end
      mask Callback h_Data_Rotor_Back_M:
      | if length(get_param(gcb,'h_Data_Rotor_Back_M')) == 2 %on
      |     set_param(gcb,'h_Eqn_Rotor_Back_M','off');
      |     set_param(gcb,'h_Const_Rotor_Back_M','off');
      |     MSK_SEC_Enables2_TMATS('h_Data_Rotor_Back_M',[56 57],'dis')
      |     MSK_SEC_Enables2_TMATS('h_Data_Rotor_Back_M',[58 59 60 61 62 122],'en')
      | end
      mask Callback alpha_TempDependence_Rotor_M:
      | MSK_SEC_Enables_TMATS('alpha_TempDependence_Rotor_M',65,'dis')
      | MSK_SEC_Enables_TMATS('alpha_TempDependence_Rotor_M',[66 67],'en')
      mask Callback E_TempDependence_Rotor_M:
      | MSK_SEC_Enables_TMATS('E_TempDependence_Rotor_M',69,'dis')
      | MSK_SEC_Enables_TMATS('E_TempDependence_Rotor_M',[70 71],'en')
      mask Callback v_TempDependence_Rotor_M:
      | MSK_SEC_Enables_TMATS('v_TempDependence_Rotor_M',73,'dis')
      | MSK_SEC_Enables_TMATS('v_TempDependence_Rotor_M',[74 75],'en')
      mask Callback k_TempDependence_Case_M:
      | MSK_SEC_Enables_TMATS('k_TempDependence_Case_M',82,'dis')
      | MSK_SEC_Enables_TMATS('k_TempDependence_Case_M',[83 84],'en')
      mask Callback Cp_TempDependence_Case_M:
      | MSK_SEC_Enables_TMATS('Cp_TempDependence_Case_M',86,'dis')
      | MSK_SEC_Enables_TMATS('Cp_TempDependence_Case_M',[87 88],'en')
      mask Callback h_Const_Case_In_M:
      | if length(get_param(gcb,'h_Const_Case_In_M')) == 2 %on
      |     set_param(gcb,'h_Eqn_Case_In_M','off');
      |     set_param(gcb,'h_Data_Case_In_M','off');
      |     MSK_SEC_Enables2_TMATS('h_Const_Case_In_M',92,'en')
      |     MSK_SEC_Enables2_TMATS('h_Const_Case_In_M',[93 94 95 96 97 98 124],'dis')
      | end
      mask Callback h_Eqn_Case_In_M:
      | if length(get_param(gcb,'h_Eqn_Case_In_M')) == 2 %on
      |     set_param(gcb,'h_Const_Case_In_M','off');
      |     set_param(gcb,'h_Data_Case_In_M','off');
      |     MSK_SEC_Enables2_TMATS('h_Eqn_Case_In_M',[93 94 95 124],'en')
      |     MSK_SEC_Enables2_TMATS('h_Eqn_Case_In_M',[92 96 97 98],'dis')
      | end
      mask Callback h_Data_Case_In_M:
      | if length(get_param(gcb,'h_Data_Case_In_M')) == 2 %on
      |     set_param(gcb,'h_Eqn_Case_In_M','off');
      |     set_param(gcb,'h_Const_Case_In_M','off');
      |     MSK_SEC_Enables2_TMATS('h_Data_Case_In_M',[92 93],'dis')
      |     MSK_SEC_Enables2_TMATS('h_Data_Case_In_M',[94 95 96 97 98 124],'en')
      | end
      mask Callback h_Const_Case_Out_M:
      | if length(get_param(gcb,'h_Const_Case_Out_M')) == 2 %on
      |     set_param(gcb,'h_Eqn_Case_Out_M','off');
      |     set_param(gcb,'h_Data_Case_Out_M','off');
      |     MSK_SEC_Enables2_TMATS('h_Const_Case_Out_M',102,'en')
      |     MSK_SEC_Enables2_TMATS('h_Const_Case_Out_M',[103 104 105 106 107 108 126],'dis')
      | end
      mask Callback h_Eqn_Case_Out_M:
      | if length(get_param(gcb,'h_Eqn_Case_Out_M')) == 2 %on
      |     set_param(gcb,'h_Const_Case_Out_M','off');
      |     set_param(gcb,'h_Data_Case_Out_M','off');
      |     MSK_SEC_Enables2_TMATS('h_Eqn_Case_Out_M',[103 104 105 126],'en')
      |     MSK_SEC_Enables2_TMATS('h_Eqn_Case_Out_M',[102 106 107 108],'dis')
      | end
      mask Callback h_Data_Case_Out_M:
      | if length(get_param(gcb,'h_Data_Case_Out_M')) == 2 %on
      |     set_param(gcb,'h_Eqn_Case_Out_M','off');
      |     set_param(gcb,'h_Const_Case_Out_M','off');
      |     MSK_SEC_Enables2_TMATS('h_Data_Case_Out_M',[102 103],'dis')
      |     MSK_SEC_Enables2_TMATS('h_Data_Case_Out_M',[104 105 106 107 108 126],'en')
      | end
      mask Callback alpha_TempDependence_Case_M:
      | MSK_SEC_Enables_TMATS('alpha_TempDependence_Case_M',112,'dis')
      | MSK_SEC_Enables_TMATS('alpha_TempDependence_Case_M',[113 114],'en')
      mask DialogControl Container18 Prompt: Heat capacity
      mask DialogControl Container36 Prompt: Model Selection
      mask DialogControl Container33 Prompt: Thermal Expansion Coefficient
      mask DialogControl Container37 Prompt: Young's Modulus
      mask DialogControl Container25 Prompt: Material properties
      mask DialogControl Container26 Prompt: Thermal conductivity
      mask DialogControl Container28 Prompt: Heat capacity
      mask DialogControl Container38 Prompt: Thermal expansion coefficient
      mask DialogControl Container40 Prompt: Young's Modulus
      mask DialogControl Container41 Prompt: Poisson's Ratio
      mask DialogControl Container75 Prompt: Material Parameters
      mask DialogControl Container76 Prompt: Thermal conductivity
      mask DialogControl Container78 Prompt: Heat Capacity
      mask DialogControl Container83 Prompt: Thermal Expansion Coefficient
      mask DialogControl Container67 Prompt: Core flow
      mask DialogControl Container68 Prompt: Cooling flows
  Steady-State Tip Clearance : Subsystem  mask(TCML - Steady-State Tip Clearance Library Block){eta_Blade_M=0.5, T0_Blade_M=1800, h_Const_Blade_M=off, h_Eqn_Blade_M=on, h_Data_Blade_M=off, h_Blade_M=0.03, hcoeff_Blade_M=0.03, Wdes_Blade_M=3, Tdes_Blade_M=1800, Wc_Blade_Data_M=[0 100], Tc_Blade_Data_M=[0 10], h_Blade_Data_M=[0.03 0.03; 0.03 0.03], L_Blade_M=0.125, rho_Blade_M=15.8975, alpha_TempDependence_Blade_M=on, alpha_Blade_M=0.000008, Talpha_Blade_Data_M=[0 10000], alpha_Blade_Data_M=[0.000008 0.000008], E_TempDependence_Blade_M=on, E_Blade_M=3974400000, TE_Blade_Data_M=[0 10000], E_Blade_Data_M=[3974400000 3974400000], W_Rotor_M=0.0833, n_Rotor_M=20, T0_Rotor_M=700*ones(1,20), rho_Rotor_M=15.8975, k_TempDependence_Rotor_M=on, k_Rotor_M=0.0015, Tk_Rotor_Data_M=[0 10000], k_Rotor_Data_M=[0.0015 0.0015], h_Const_Rotor_Front_M=off, h_Eqn_Rotor_Front_M=on, h_Data_Rotor_Front_M=off, h_Rotor_Front_M=0.03, hcoeff_Rotor_Front_M=0.03, Wdes_Rotor_Front_M=1, Tdes_Rotor_Front_M=700, Wc_Rotor_Front_Data_M=[0 100], Tc_Rotor_Front_Data_M=[0 10], h_Rotor_Front_Data_M=[0.003 0.003; 0.003 0.003], h_Const_Rotor_Back_M=off, h_Eqn_Rotor_Back_M=on, h_Data_Rotor_Back_M=off, h_Rotor_Back_M=0.03, hcoeff_Rotor_Back_M=0.03, Wdes_Rotor_Back_M=1, Tdes_Rotor_Back_M=700, Wc_Rotor_Back_Data_M=[0 100], Tc_Rotor_Back_Data_M=[0 10], h_Rotor_Back_Data_M=[0.003 0.003; 0.003 0.003], Ro_Rotor_M=1, alpha_TempDependence_Rotor_M=on, alpha_Rotor_M=0.000008, Talpha_Rotor_Data_M=[0 10000], alpha_Rotor_Data_M=[0.000008 0.000008], E_TempDependence_Rotor_M=on, E_Rotor_M=3974400000, TE_Rotor_Data_M=[0 10000], E_Rotor_Data_M=[3974400000 3974400000], v_TempDependence_Rotor_M=on, v_Rotor_M=0.3, Tv_Rotor_Data_M=[0 10000], v_Rotor_Data_M=[0.3 0.3], W_Case_M=0.0156, n_Case_M=20, T0_Case_M=1000*ones(1,20), rho_Case_M=15.8975, k_TempDependence_Case_M=on, k_Case_M=0.0015, Tk_Case_Data_M=[0 10000], k_Case_Data_M=[0.0015 0.0015], h_Const_Case_In_M=off, h_Eqn_Case_In_M=on, h_Data_Case_In_M=off, h_Case_In_M=0.02, hcoeff_Case_In_M=0.02, Wdes_Case_In_M=3, Tdes_Case_In_M=1000, Wc_Case_In_Data_M=[0 100], Tc_Case_In_Data_M=[1 10], h_Case_In_Data_M=[0.02 0.02; 0.02 0.02], h_Const_Case_Out_M=off, h_Eqn_Case_Out_M=on, h_Data_Case_Out_M=off, h_Case_Out_M=0.01, hcoeff_Case_Out_M=0.01, Wdes_Case_Out_M=1, Tdes_Case_Out_M=1000, Wc_Case_Out_Data_M=[0 100], Tc_Case_Out_Data_M=[0 10], h_Case_Out_Data_M=[0.01 0.01; 0.01 0.01], Ri_Case_M=1.1344, L_Shroud_M=1/12, alpha_TempDependence_Case_M=on, alpha_Case_M=0.000008, Talpha_Case_Data_M=[0 10000], alpha_Case_Data_M=[0.000008 0.000008]}
      mask prompts: eta_Blade_M "eta_Blade_M - Film cooling coefficient [1x1]"; T0_Blade_M "T0_Blade_M - Initial temperature of the blade (R) [1x1]"; h_Const_Blade_M "h_Const_Blade_M - Constant convective heat transfer coefficient (Btu/(sec-ft^2-R)) [1x1]"; h_Eqn_Blade_M "h_Eqn_Blade_M - h = hcoeff*(T/Tdes)^0.23*(W/Wdes)^0.8 [1x1]"; h_Data_Blade_M "h_Data_Blade_M - h = f(T/Tdes, W/Wdes) based on data [1x1]"; h_Blade_M "h_Blade_M - Constant convective heat transfer coefficient (Btu/(sec-ft^2-R)) [1x1]"; hcoeff_Blade_M "hcoeff_Blade_M - Coefficient in the convective heat transfer coefficient model h = hcoeff*(T/Tdes)^0.23*(W/Wdes)^0.8 [1x1]"; Wdes_Blade_M "Wdes_Blade_M - Design mass flow rate of core flow for a known convective heat transfer coefficient (slug/sec) [1x1]"; Tdes_Blade_M "Tdes_Blade_M - Design temperature of core flow for a known convective heat transfer coefficient (Btu/(slug-R)) [1x1]"; Wc_Blade_Data_M "Wc_Blade_Data_M - Non-dimensional mass flow rate (W/Wdes) data array for determining the convective heat transfer coefficient [bx1]"; Tc_Blade_Data_M "Tc_Blade_Data_M - Non-dimensional temperature (T/Tdes) array for determining the convective heat transfer coefficient [cx1]"; h_Blade_Data_M "h_Blade_Data_M - Matrix of convective heat transfer coefficients with rows corresponding to W/Wdes and columns corresponding to T/Tdes (Btu/(sec-ft^2-R)) [bxc]"; L_Blade_M "L_Blade_M - Blade length (ft) [1x1]"; rho_Blade_M "rho_Blade_M - Blade density (slug/ft^3) [1x1]"; alpha_TempDependence_Blade_M "alpha_TempDependence_Blade_M - Thermal expansion coefficient temperature dependence (unchecked - alpha = constant, checked - alpha is temperature dependent)"; alpha_Blade_M "alpha_Blade_M - Constant thermal expansion coefficient (1/R) [1x1]"; Talpha_Blade_Data_M "Talpha_Blade_Data_M - Temperature array for interpolating the thermal expansion coefficient (R) [dx1]"; alpha_Blade_Data_M "alpha_Blade_Data_M - Thermal expansion coefficient array for interpolating the thermal expansion coefficient (1/R) [dx1]"; E_TempDependence_Blade_M "E_TempDependence_Blade_M - Young's Modulus temperature dependence (unchecked - E = constant, checked - E is temperature dependent)"; E_Blade_M "E_Blade_M - Constant Young's Modulus (lbf/ft^2) [1x1]"; TE_Blade_Data_M "TE_Blade_Data_M - Temperature array for interpolating Young's Modulus (R) [ex1]"; E_Blade_Data_M "E_Blade_Data_M - Young's Modulus array for interpolating Young's Modulus (lbf/ft^2) [ex1]"; W_Rotor_M "W_Rotor_M - Width of the rotor (ft) [1x1]"; n_Rotor_M "n_Rotor_M - Number of nodes in spatial discretization [1x1]"; T0_Rotor_M "T0_Rotor_M - Intial temperature array (R) [n_Rotor_Mx1]"; rho_Rotor_M "rho_Rotor_M - Rotor density (slug/ft^3) [1x1]"; k_TempDependence_Rotor_M "k_TempDependence_Rotor_M - Thermal conductivity temperature dependence (unchecked - k = constant, checked - k is temperature dependent)"; k_Rotor_M "k_Rotor_M - Constant thermal conductivity (Btu/(sec-ft-R)) [1x1]"; Tk_Rotor_Data_M "Tk_Rotor_Data_M - Temperature array for interpolating the thermal conductivity (R) [fx1]"; k_Rotor_Data_M "k_Rotor_Data_M - Thermal conductivity array for interpolating the thermal conductivity (Btu/(sec-ft-R)) [fx1]"; h_Const_Rotor_Front_M "h_Const_Rotor_Front_M - Constant convective heat transfer coefficient (Btu/(sec-ft^2-R))"; h_Eqn_Rotor_Front_M "h_Eqn_Rotor_Front_M - h = hcoeff*(T/Tdes)^0.23*(W/Wdes)^0.8"; h_Data_Rotor_Front_M "h_Data_Rotor_Front_M = h = f(T/Tdes, W/Wdes) based on data"; h_Rotor_Front_M "h_Rotor_Front_M - Constant convective heat transfer coefficient (Btu/(sec-ft^2-R)) [1x1]"; hcoeff_Rotor_Front_M "hcoeff_Rotor_Front_M - Coefficient in the convective heat transfer coefficient model h = hcoeff*(T/Tdes)^0.23*(W/Wdes)^0.8 [1x1]"; Wdes_Rotor_Front_M "Wdes_Rotor_Front_M - Design mass flow rate of core flow for a known convective heat transfer coefficient (slug/sec) [1x1]"; Tdes_Rotor_Front_M "Tdes_Rotor_Front_M - Design temperature of core flow for a known convective heat transfer coefficient (Btu/(slug-R)) [1x1]"; Wc_Rotor_Front_Data_M "Wc_Rotor_Front_Data_M - Non-dimensional mass flow rate (W/Wdes) data array for determining the convective heat transfer coefficient [hx1]"; Tc_Rotor_Front_Data_M "Tc_Rotor_Front_Data_M - Non-dimensional temperature (T/Tdes) array for determining the convective heat transfer coefficient [ix1]"; h_Rotor_Front_Data_M "h_Rotor_Front_Data_M - Matrix of convective heat transfer coefficients with rows corresponding to W/Wdes and columns corresponding to T/Tdes (Btu/(sec-ft^2-R)) [hxi]"; h_Const_Rotor_Back_M "h_Const_Rotor_Back_M - Constant convective heat transfer coefficient (Btu/(sec-ft^2-R))"; h_Eqn_Rotor_Back_M "h_Eqn_Rotor_Back_M - h = hcoeff*(T/Tdes)^0.23*(W/Wdes)^0.8"; h_Data_Rotor_Back_M "h_Data_Rotor_Back_M - h = f(T/Tdes, W/Wdes) based on data"; h_Rotor_Back_M "h_Rotor_Back_M - Constant convective heat transfer coefficient (Btu/(sec-ft^2-R)) [1x1]"; hcoeff_Rotor_Back_M "hcoeff_Rotor_Back_M - Coefficient in the convective heat transfer coefficient model h = hcoeff*(T/Tdes)^0.23*(W/Wdes)^0.8 [1x1]"; Wdes_Rotor_Back_M "Wdes_Rotor_Back_M - Design mass flow rate of core flow for a known convective heat transfer coefficient (slug/sec) [1x1]"; Tdes_Rotor_Back_M "Tdes_Rotor_Back_M - Design temperature of core flow for a known convective heat transfer coefficient (Btu/(slug-R)) [1x1]"; Wc_Rotor_Back_Data_M "Wc_Rotor_Back_Data_M - Non-dimensional mass flow rate (W/Wdes) data array for determining the convective heat transfer coefficient [jx1]"; Tc_Rotor_Back_Data_M "Tc_Rotor_Back_Data_M - Non-dimensional temperature (T/Tdes) array for determining the convective heat transfer coefficient [kx1]"; h_Rotor_Back_Data_M "h_Rotor_Back_Data_M - Matrix of convective heat transfer coefficients with rows corresponding to W/Wdes and columns corresponding to T/Tdes (Btu/(sec-ft^2-R)) [jxk]"; Ro_Rotor_M "Ro_Rotor_M - Outer radius of the rotor (ft) [1x1]"; alpha_TempDependence_Rotor_M "alpha_TempDependence_Rotor_M - Thermal expansion coefficient temperature dependence (unchecked - alpha = constant, checked - alpha is temperature dependent)"; alpha_Rotor_M "alpha_Rotor_M - Constant thermal expansion coefficient (1/R) [1x1]"; Talpha_Rotor_Data_M "Talpha_Rotor_Data_M - Temperature array for interpolating the thermal expansion coefficient (R) [lx1]"; alpha_Rotor_Data_M "alpha_Rotor_Data_M - Thermal expansion coefficient array for interpolating the thermal expansion coefficient (1/R) [lx1]"; E_TempDependence_Rotor_M "E_TempDependence_Rotor_M - Young's Modulus temperature dependence (uncheck - E = constant, checked - E is temperature dependent)"; E_Rotor_M "E_Rotor_M - Constant Young's Modulus (lbf/ft^2) [1x1]"; TE_Rotor_Data_M "TE_Rotor_Data_M - Temperature array for interpolating Young's Modulus (R) [mx1]"; E_Rotor_Data_M "E_Rotor_Data_M - Young's Modulus array for interpolating Young's Modulus (lbf/ft^2) [mx1]"; v_TempDependence_Rotor_M "v_TempDependence_Rotor_M - Poisson's Ratio temperature dependence"; v_Rotor_M "v_Rotor_M - Constant Poisson's ratio [1x1]"; Tv_Rotor_Data_M "Tv_Rotor_Data_M - Temperature array for interpolating Poisson's ratio (R) [nx1]"; v_Rotor_Data_M "v_Rotor_Data_M - Poisson's ratio array for interpolating Poisson's ratio [nx1]"; W_Case_M "W_Case_M - Width of the case (ft) [1x1]"; n_Case_M "n_Case_M - Number of nodes in the spatial discretization [1x1]"; T0_Case_M "T0_Case_M - Initial temperature array (R) [(n_Case_M)x1]"; rho_Case_M "rho_Case_M - Density (slug/ft^3) [1x1]"; k_TempDependence_Case_M "k_TempDependence_Case_M - Thermal conductivity temperature dependence (unchecked - k = constant, checked - k is temperature dependent)"; k_Case_M "k_Case_M - Constant thermal conductivity (Btu/(sec-ft-R)) [1x1]"; Tk_Case_Data_M "Tk_Case_Data_M - Temperature array for interpolating thermal conductivity (R) [ox1]"; k_Case_Data_M "k_Case_Data_M - Thermal conductivity array for interpolating thermal conductivity (Btu/(sec-ft-R)) [ox1]"; h_Const_Case_In_M "h_Const_Case_In_M - Constant convective heat transfer coefficient (Btu/(sec-ft^2-R))"; h_Eqn_Case_In_M "h_Eqn_Case_In_M - h = hcoeff*(T/Tdes)^0.23*(W/Wdes)^0.8"; h_Data_Case_In_M "h_Data_Case_In_M - h = f(T/Tdes, W/Wdes) based on data"; h_Case_In_M "h_Case_In_M - Codnstant convective heat transfer coefficient (Btu/(sec-ft^2-R)) [1x1]"; hcoeff_Case_In_M "hcoeff_Case_In_M - Coefficient in the convective heat transfer coefficient model h = hcoeff*(T/Tdes)^0.23*(W/Wdes)^0.8 [1x1]"; Wdes_Case_In_M "Wdes_Case_In_M - Design mass flow rate of core flow for a known convective heat transfer coefficient (slug/sec) [1x1]"; Tdes_Case_In_M "Tdes_Case_In_M - Design temperature of core flow for a known convective heat transfer coefficient (Btu/(slug-R)) [1x1]"; Wc_Case_In_Data_M "Wc_Case_In_Data_M - Non-dimensional mass flow rate (W/Wdes) data array for determining the convective heat transfer coefficient [sx1]"; Tc_Case_In_Data_M "Tc_Case_In_Data_M - Non-dimensional temperature (T/Tdes) array for determining the convective heat transfer coefficient [tx1]"; h_Case_In_Data_M "h_Case_In_Data_M - Matrix of convective heat transfer coefficients with rows corresponding to W/Wdes and columns corresponding to T/Tdes (Btu/(sec-ft^2-R)) [sxt]"; h_Const_Case_Out_M "h_Const_Case_Out_M - Constant convective heat transfer coefficient (Btu/(sec-ft^2-R))"; h_Eqn_Case_Out_M "h_Eqn_Case_Out_M - h = hcoeff*(T/Tdes)^0.23*(W/Wdes)^0.8"; h_Data_Case_Out_M "h_Data_Case_Out_M - h = f(T/Tdes, W/Wdes) based on data"; h_Case_Out_M "h_Case_Out_M - Codnstant convective heat transfer coefficient (Btu/(sec-ft^2-R)) [1x1]"; hcoeff_Case_Out_M "hcoeff_Case_Out_M - Coefficient in the convective heat transfer coefficient model h = hcoeff*(T/Tdes)^0.23*(W/Wdes)^0.8 [1x1]"; Wdes_Case_Out_M "Wdes_Case_Out_M - Design mass flow rate of core flow for a known convective heat transfer coefficient (slug/sec) [1x1]"; Tdes_Case_Out_M "Tdes_Case_Out_M - Design temperature of core flow for a known convective heat transfer coefficient (Btu/(slug-R)) [1x1]"; Wc_Case_Out_Data_M "Wc_Case_Out_Data_M - Non-dimensional mass flow rate (W/Wdes) data array for determining the convective heat transfer coefficient [ux1]"; Tc_Case_Out_Data_M "Tc_Case_Out_Data_M - Non-dimensional temperature (T/Tdes) array for determining the convective heat transfer coefficient [vx1]"; h_Case_Out_Data_M "h_Case_Out_Data_M - Matrix of convective heat transfer coefficients with rows corresponding to W/Wdes and columns corresponding to T/Tdes (Btu/(sec-ft^2-R)) [uxv]"; Ri_Case_M "Ri_Case_M - Inner radius of the case (ft) [1x1]"; L_Shroud_M "L_Shroud_M - Distrance between the inner surface of the shroud and inner surface of the case (ft) [1x1]"; alpha_TempDependence_Case_M "alpha_TempDependence_Case_M - Thermal expansion coefficient temperature dependence (unchecked - alpha = constant, checked - alpha is temperature dependent)"; alpha_Case_M "alpha_Case_M - Constant thermal expansion coefficient (1/R) [1x1]"; Talpha_Case_Data_M "Talpha_Case_Data_M - Temperature array for interpolating the thermal expansion coefficient (R) [wx1]"; alpha_Case_Data_M "alpha_Case_Data_M - Thermal expansion coefficient array for interpolating the thermal expansion coefficient (1/R) [wx1]"
      mask help:
      | This block produces the steady-state tip clearance solution for a given operating condition. That is to say that it provides the tip clearance and relavant temperatures and lengths of components once all dynamics have resided. This block is useful for initializing the dynamic tip clearance blocks in this library as well as evaluating steady-state tip clearance and engine performance impact on-the-fly.
      |
      | This function approximates axisymmetric tip clearance variation inside turbomachinery (i.e. compressors and turbines). It models the deformation of the rotor, blade, and shroud (containment structure) due to elastic thermal and centrifugal deformation. The blade is modeled as a lumped mass and the rotor and shroud use a 1-D finite difference approach for temperature determination. The thermal deformation models use the average component temperature. This function has numerous options for modeling convective heat transfer coefficients and temperature dependence of various parameters including thermal conductivity, heat capacity, thermal expansion coefficient, Young's Modulus, and Poisson's ratio. If temperature dependent thermal properties are specified then the average temperature of the component is calculated, the thermal property is chosen based on the average temperature, the steady-state solution is evaluated with this constant thermal property value, and the solution is iterated on until it converges.
      |
      | Units of the inputs and parameters are indicated so be sure to abide by them. Dimensions are indicated for the parameters and all inputs are scalars. See the block help menu for more details.
      mask init:
      | % check for warning/errors -----------------------------------------------%
      | 
      | % Blade -----------------------------%
      | 
      | % eta_Blade_M
      | if length(eta_Blade_M) ~= 1
      |     fprintf('warning in %s: eta_Blade_M must be a scalar entry.\n',gcb)
      | end
      | if eta_Blade_M < 0 || eta_Blade_M > 1
      |     fprintf('warning in %s: eta_Blade_M must be between 0 and 1.\n',gcb)
      | end
      | 
      | % T0_Blade_M
      | if length(T0_Blade_M) ~= 1
      |     fprintf('warning in %s: T0_Blade_M must be a scalar entry.\n',gcb)
      | end
      | if T0_Blade_M < 0 || isreal(T0_Blade_M) == 0
      |     fprintf('warning in %s: T0_Blade_M must be a real positive number.\n',gcb)
      | end
      | 
      | % h_Blade_M
      | if length(h_Blade_M) ~= 1
      |     fprintf('warning in %s: h_Blade_M must be a scalar.\n',gcb)
      | end
      | if h_Blade_M < 0 || isreal(h_Blade_M) == 0
      |     fprintf('warning in %s: h_Blade_M must be a real positive entry.\n',gcb)
      | end
      | 
      | % hcoeff_Blade_M
      | if length(hcoeff_Blade_M) ~= 1
      |     fprintf('warning in %s: hcoeff_Blade_M must be a scalar.\n',gcb)
      | end
      | if hcoeff_Blade_M < 0 || isreal(hcoeff_Blade_M) == 0
      |     fprintf('warning in %s: hcoeff_Blade_M must be a real positive entry.\n',gcb)
      | end
      | 
      | % Wdes_Blade_M
      | if length(Wdes_Blade_M) ~= 1
      |     fprintf('warning in %s: Wdes_Blade_M must be a scalar entry.\n',gcb)
      | end
      | if Wdes_Blade_M <= 0 || isreal(Wdes_Blade_M) == 0
      |     fprintf('warning in %s: Wdes_Blade_M must be a real positive number.\n',gcb)
      | end
      | 
      | % Tdes_Blade_M
      | if length(Tdes_Blade_M) ~= 1
      |     fprintf('warning in %s: Tdes_Blade_M must be a scalar entry.\n',gcb)
      | end
      | if Tdes_Blade_M <= 0 || isreal(Tdes_Blade_M) == 0
      |     fprintf('warning in %s: Tdes_Blade_M must be a real positive number.\n',gcb)
      | end
      | 
      | % Wc_Blade_Data_M, Tc_Blade_Data_M & h_Blade_Data_M
      | [nR, nC] = size(h_Blade_Data_M);
      | if nR < 2 || nC < 2
      |     fprintf('warning in %s: h_Blade_Data_M must be a matrix of at least 2 rows and 2 columns.\n',gcb)
      | end
      | if length(Wc_Blade_Data_M) ~= nR
      |     fprintf('warning in %s: Wc_Blade_Data_M must have the same number of elements as rows in h_Blade_Data_M.\n',gcb)
      | end
      | if length(Tc_Blade_Data_M) ~= nC
      |     fprintf('warning in %s: Tc_Blade_Data_M must have the same number of elements as columns in h_Blade_Data_M.\n',gcb)
      | end
      | real_Wc_Blade_Data_M = isreal(Wc_Blade_Data_M);
      | if min(real_Wc_Blade_Data_M) == 0
      |     fprintf('warning in %s: Wc_Blade_Data_M must have all real entries.\n',gcb)
      | end
      | diff_Wc_Blade_Data_M = diff(Wc_Blade_Data_M);
      | if min(diff_Wc_Blade_Data_M) <= 0
      |     fprintf('warning in %s: Wc_Blade_Data_M must be monotonically increasing.\n',gcb)
      | end
      | real_Tc_Blade_Data_M = isreal(Tc_Blade_Data_M);
      | if min(real_Tc_Blade_Data_M) == 0
      |     fprintf('warning in %s: Tc_Blade_Data_M must have all real entries.\n',gcb)
      | end
      | diff_Tc_Blade_Data_M = diff(Tc_Blade_Data_M);
      | if min(diff_Tc_Blade_Data_M) <= 0
      |     fprintf('warning in %s: Tc_Blade_Data_M must be monotonically increasing.\n',gcb)
      | end
      | if min(Tc_Blade_Data_M) < 0
      |     fprintf('warning in %s: Elements of Tc_Blade_Data_M are less than 0 which is impossible.\n',gcb)
      | end
      | real_h_Blade_Data_M = isreal(h_Blade_Data_M);
      | if min(real_h_Blade_Data_M) == 0 || min(min(h_Blade_Data_M)) < 0
      |     fprintf('warning in %s: h_Blade_Data_M must have all real positive entries.\n',gcb)
      | end
      | 
      | % L_Blade_M
      | if length(L_Blade_M) ~= 1
      |     fprintf('warning in %s: L_Blade_M must be a scalar entry.\n',gcb)
      | end
      | if L_Blade_M <= 0 || isreal(L_Blade_M) == 0
      |     fprintf('warning in %s: L_Blade_M must be a real positive number.\n',gcb)
      | end
      | 
      | % rho_Blade_M
      | if length(rho_Blade_M) ~= 1
      |     fprintf('warning in %s: rho_Blade_M must be a scalar entry.\n',gcb)
      | end
      | if rho_Blade_M <= 0 || isreal(rho_Blade_M) == 0
      |     fprintf('warning in %s: rho_Blade_M must be a real positive number.\n',gcb)
      | end
      | 
      | % E_Blade_M
      | if length(E_Blade_M) ~= 1
      |     fprintf('warning in %s: E_Blade_M must be a scalar entry.\n',gcb)
      | end
      | if E_Blade_M <= 0 || isreal(E_Blade_M) == 0
      |     fprintf('warning in %s: E_Blade_M must be a real positive number.\n',gcb)
      | end
      | 
      | % TE_Blade_Data_M & E_Blade_Data_M
      | if length(TE_Blade_Data_M) < 2
      |     fprintf('warning in %s: TE_Blade_Data_M must have at least 2 elements.\n',gcb)
      | end
      | if length(E_Blade_Data_M) < 2
      |     fprintf('warning in %s: E_Blade_Data_M must have at least 2 elements.\n',gcb)
      | end
      | if length(TE_Blade_Data_M) ~= length(E_Blade_Data_M)
      |     fprintf('warning in %s: TE_Blade_Data_M and E_Blade_Data_M must have the same dimensions.\n',gcb)
      | end
      | real_TE_Blade_Data_M = isreal(TE_Blade_Data_M);
      | if min(real_TE_Blade_Data_M) == 0
      |     fprintf('warning in %s: TE_Blade_Data_M must have all real entries.\n',gcb)
      | end
      | diff_TE_Blade_Data_M = diff(TE_Blade_Data_M);
      | if min(diff_TE_Blade_Data_M) <= 0
      |     fprintf('warning in %s: TE_Blade_Data_M must be monotonically increasing.\n',gcb)
      | end
      | if min(TE_Blade_Data_M) < 0
      |     fprintf('warning in %s: Elements of TE_Blade_Data_M are below 0 which is theoretically impossible.\n',gcb)
      | end
      | real_E_Blade_Data_M = isreal(E_Blade_Data_M);
      | if min(real_E_Blade_Data_M) == 0
      |     fprintf('warning in %s: E_Blade_Data_M must have all real entries.\n',gcb)
      | end
      | if min(E_Blade_Data_M) <= 0
      |     fprintf('warning in %s: Elements of E_Blade_Data_M are below 0 which is impossible.\n',gcb)
      | end
      | 
      | % Blade variables checked by underlying blocks:
      | %   alpha_Blade_M
      | %   Talpha_Blade_Data_M
      | %   alpha_Blade_Data_M
      | 
      | % Rotor --------------------------%
      | 
      | % W_Rotor_M
      | if length(W_Rotor_M) ~= 1
      |     fprintf('warning in %s: W_Rotor_M must be a scalar entry.\n',gcb)
      | end
      | if W_Rotor_M <= 0 || isreal(W_Rotor_M) == 0
      |     fprintf('warning in %s: W_Rotor_M must be a real positive number.\n',gcb)
      | end
      | 
      | % n_Rotor_M
      | if length(n_Rotor_M) ~= 1
      |     fprintf('warning in %s: n_Rotor_M must be a scalar entry.\n',gcb)
      | end
      | if n_Rotor_M <= 0 || isreal(n_Rotor_M) == 0
      |     fprintf('warning in %s: n_Rotor_M must be a real positive number.\n',gcb)
      | end
      | if n_Rotor_M < 4
      |     fprintf('warning in %s: n_Rotor_M must be >= 4.\n',gcb)
      | end
      | 
      | % T0_Rotor_M
      | if length(T0_Rotor_M) ~= n_Rotor_M
      |     fprintf('warning in %s: T0_Rotor_M must be an array with n_Rotor_M elements.\n',gcb)
      | end
      | real_T0_Rotor_M = isreal(T0_Rotor_M);
      | if min(T0_Rotor_M) <= 0 || min(real_T0_Rotor_M) == 0
      |     fprintf('warning in %s: T0_Rotor_M must have all real positive entries.\n',gcb)
      | end
      | 
      | % rho_Rotor_M
      | if length(rho_Rotor_M) ~= 1
      |     fprintf('warning in %s: rho_Rotor_M must be a scalar entry.\n',gcb)
      | end
      | if rho_Rotor_M <= 0 || isreal(rho_Rotor_M) == 0
      |     fprintf('warning in %s: rho_Rotor_M must be a real positive number.\n',gcb)
      | end
      | 
      | % k_Rotor_M
      | if length(k_Rotor_M) ~= 1
      |     fprintf('warning in %s: k_Rotor_M must be a scalar entry.\n',gcb)
      | end
      | if k_Rotor_M <= 0 || isreal(k_Rotor_M) == 0
      |     fprintf('warning in %s: k_Rotor_M must be a real positive number.\n',gcb)
      | end
      | 
      | % Tk_Rotor_Data_M & k_Rotor_Data_M
      | if length(Tk_Rotor_Data_M) < 2
      |     fprintf('warning in %s: Tk_Rotor_Data_M must have at least 2 elements.\n',gcb)
      | end
      | if length(k_Rotor_Data_M) < 2
      |     fprintf('warning in %s: k_Rotor_Data_M must have at least 2 elements.\n',gcb)
      | end
      | if length(Tk_Rotor_Data_M) ~= length(k_Rotor_Data_M)
      |     fprintf('warning in %s: Tk_Rotor_Data_M and k_Rotor_Data_M must have the same dimensions.\n',gcb)
      | end
      | real_Tk_Rotor_Data_M = isreal(Tk_Rotor_Data_M);
      | if min(real_Tk_Rotor_Data_M) == 0
      |     fprintf('warning in %s: Tk_Rotor_Data_M must have all real entries.\n',gcb)
      | end
      | diff_Tk_Rotor_Data_M = diff(Tk_Rotor_Data_M);
      | if min(diff_Tk_Rotor_Data_M) <= 0
      |     fprintf('warning in %s: Tk_Rotor_Data_M must be monotonically increasing.\n',gcb)
      | end
      | if min(Tk_Rotor_Data_M) < 0
      |     fprintf('warning in %s: Elements of Tk_Rotor_Data_M are below 0 which is theoretically impossible.\n',gcb)
      | end
      | real_k_Rotor_Data_M = isreal(k_Rotor_Data_M);
      | if min(real_k_Rotor_Data_M) == 0
      |     fprintf('warning in %s: k_Rotor_Data_M must have all real entries.\n',gcb)
      | end
      | if min(k_Rotor_Data_M) <= 0
      |     fprintf('warning in %s: Elements of k_Rotor_Data_M are below 0 which is impossible.\n',gcb)
      | end
      | 
      | % hcoeff_Rotor_Front_M
      | if length(hcoeff_Rotor_Front_M) ~= 1
      |     fprintf('warning in %s: hcoeff_Rotor_Front_M must be a scalar.\n',gcb)
      | end
      | if hcoeff_Rotor_Front_M < 0 || isreal(hcoeff_Rotor_Front_M) == 0
      |     fprintf('warning in %s: hcoeff_Rotor_Front_M must be a real positive entry.\n',gcb)
      | end
      | 
      | % Wdes_Rotor_Front_M
      | if length(Wdes_Rotor_Front_M) ~= 1
      |     fprintf('warning in %s: Wdes_Rotor_Front_M must be a scalar entry.\n',gcb)
      | end
      | if Wdes_Rotor_Front_M <= 0 || isreal(Wdes_Rotor_Front_M) == 0
      |     fprintf('warning in %s: Wdes_Rotor_Front_M must be a real positive number.\n',gcb)
      | end
      | 
      | % Tdes_Rotor_Front_M
      | if length(Tdes_Rotor_Front_M) ~= 1
      |     fprintf('warning in %s: Tdes_Rotor_Front_M must be a scalar entry.\n',gcb)
      | end
      | if Tdes_Rotor_Front_M <= 0 || isreal(Tdes_Rotor_Front_M) == 0
      |     fprintf('warning in %s: Tdes_Rotor_Front_M must be a real positive number.\n',gcb)
      | end
      | 
      | % Wc_Rotor_Front_Data_M, Tc_Rotor_Front_Data_M & h_Rotor_Front_Data_M
      | [nR, nC] = size(h_Rotor_Front_Data_M);
      | if nR < 2 || nC < 2
      |     fprintf('warning in %s: h_Rotor_Front_Data_M must be a matrix of at least 2 rows and 2 columns.\n',gcb)
      | end
      | if length(Wc_Rotor_Front_Data_M) ~= nR
      |     fprintf('warning in %s: Wc_Rotor_Front_Data_M must have the same number of elements as rows in h_Rotor_Front_Data_M.\n',gcb)
      | end
      | if length(Tc_Rotor_Front_Data_M) ~= nC
      |     fprintf('warning in %s: Tc_Rotor_Front_Data_M must have the same number of elements as columns in h_Rotor_Front_Data_M.\n',gcb)
      | end
      | real_Wc_Rotor_Front_Data_M = isreal(Wc_Rotor_Front_Data_M);
      | if min(real_Wc_Blade_Data_M) == 0
      |     fprintf('warning in %s: Wc_Rotor_Front_Data_M must have all real entries.\n',gcb)
      | end
      | diff_Wc_Rotor_Front_Data_M = diff(Wc_Rotor_Front_Data_M);
      | if min(diff_Wc_Rotor_Front_Data_M) <= 0
      |     fprintf('warning in %s: Wc_Rotor_Front_Data_M must be monotonically increasing.\n',gcb)
      | end
      | real_Tc_Rotor_Front_Data_M = isreal(Tc_Rotor_Front_Data_M);
      | if min(real_Tc_Rotor_Front_Data_M) == 0
      |     fprintf('warning in %s: Tc_Rotor_Front_Data_M must have all real entries.\n',gcb)
      | end
      | diff_Tc_Rotor_Front_Data_M = diff(Tc_Rotor_Front_Data_M);
      | if min(diff_Tc_Rotor_Front_Data_M) <= 0
      |     fprintf('warning in %s: Tc_Rotor_Front_Data_M must be monotonically increasing.\n',gcb)
      | end
      | if min(Tc_Blade_Data_M) < 0
      |     fprintf('warning in %s: Elements of Tc_Rotor_Front_Data_M are less than 0 which is impossible.\n',gcb)
      | end
      | real_h_Rotor_Front_Data_M = isreal(h_Rotor_Front_Data_M);
      | if min(real_h_Rotor_Front_Data_M) == 0 || min(min(h_Rotor_Front_Data_M)) < 0
      |     fprintf('warning in %s: h_Rotor_Front_Data_M must have all real positive entries.\n',gcb)
      | end
      | 
      | % hcoeff_Rotor_Back_M
      | if length(hcoeff_Rotor_Back_M) ~= 1
      |     fprintf('warning in %s: hcoeff_Rotor_Back_M must be a scalar.\n',gcb)
      | end
      | if hcoeff_Rotor_Back_M < 0 || isreal(hcoeff_Rotor_Back_M) == 0
      |     fprintf('warning in %s: hcoeff_Rotor_Back_M must be a real positive entry.\n',gcb)
      | end
      | 
      | % Wdes_Rotor_Back_M
      | if length(Wdes_Rotor_Back_M) ~= 1
      |     fprintf('warning in %s: Wdes_Rotor_Back_M must be a scalar entry.\n',gcb)
      | end
      | if Wdes_Rotor_Back_M <= 0 || isreal(Wdes_Rotor_Back_M) == 0
      |     fprintf('warning in %s: Wdes_Rotor_Back_M must be a real positive number.\n',gcb)
      | end
      | 
      | % Tdes_Rotor_Back_M
      | if length(Tdes_Rotor_Back_M) ~= 1
      |     fprintf('warning in %s: Tdes_Rotor_Back_M must be a scalar entry.\n',gcb)
      | end
      | if Tdes_Rotor_Back_M <= 0 || isreal(Tdes_Rotor_Back_M) == 0
      |     fprintf('warning in %s: Tdes_Rotor_Back_M must be a real positive number.\n',gcb)
      | end
      | 
      | % Wc_Rotor_Back_Data_M, Tc_Rotor_Back_Data_M & h_Rotor_Back_Data_M
      | [nR, nC] = size(h_Rotor_Back_Data_M);
      | if nR < 2 || nC < 2
      |     fprintf('warning in %s: h_Rotor_Back_Data_M must be a matrix of at least 2 rows and 2 columns.\n',gcb)
      | end
      | if length(Wc_Rotor_Back_Data_M) ~= nR
      |     fprintf('warning in %s: Wc_Rotor_Back_Data_M must have the same number of elements as rows in h_Rotor_Back_Data_M.\n',gcb)
      | end
      | if length(Tc_Rotor_Back_Data_M) ~= nC
      |     fprintf('warning in %s: Tc_Rotor_Back_Data_M must have the same number of elements as columns in h_Rotor_Back_Data_M.\n',gcb)
      | end
      | real_Wc_Rotor_Back_Data_M = isreal(Wc_Rotor_Back_Data_M);
      | if min(real_Wc_Rotor_Back_Data_M) == 0
      |     fprintf('warning in %s: Wc_Rotor_Back_Data_M must have all real entries.\n',gcb)
      | end
      | diff_Wc_Rotor_Back_Data_M = diff(Wc_Rotor_Back_Data_M);
      | if min(diff_Wc_Rotor_Back_Data_M) <= 0
      |     fprintf('warning in %s: Wc_Rotor_Front_Data_M must be monotonically increasing.\n',gcb)
      | end
      | real_Tc_Rotor_Back_Data_M = isreal(Tc_Rotor_Back_Data_M);
      | if min(real_Tc_Rotor_Back_Data_M) == 0
      |     fprintf('warning in %s: Tc_Rotor_Back_Data_M must have all real entries.\n',gcb)
      | end
      | diff_Tc_Rotor_Back_Data_M = diff(Tc_Rotor_Back_Data_M);
      | if min(diff_Tc_Rotor_Back_Data_M) <= 0
      |     fprintf('warning in %s: Tc_Rotor_Back_Data_M must be monotonically increasing.\n',gcb)
      | end
      | if min(Tc_Rotor_Back_Data_M) < 0
      |     fprintf('warning in %s: Elements of Tc_Rotor_Back_Data_M are less than 0 which is impossible.\n',gcb)
      | end
      | real_h_Rotor_Back_Data_M = isreal(h_Rotor_Back_Data_M);
      | if min(real_h_Rotor_Back_Data_M) == 0 || min(min(h_Rotor_Back_Data_M)) < 0
      |     fprintf('warning in %s: h_Rotor_Back_Data_M must have all real positive entries.\n',gcb)
      | end
      | 
      | % Ro_Rotor_M
      | if length(Ro_Rotor_M) ~= 1
      |     fprintf('warning in %s: Ro_Rotor_M must be a scalar entry.\n',gcb)
      | end
      | if Ro_Rotor_M <= 0 || isreal(Ro_Rotor_M) == 0
      |     fprintf('warning in %s: Ro_Rotor_M must be a real positive number.\n',gcb)
      | end
      | 
      | % E_Rotor_M
      | if length(E_Rotor_M) ~= 1
      |     fprintf('warning in %s: E_Rotor_M must be a scalar entry.\n',gcb)
      | end
      | if E_Rotor_M <= 0 || isreal(E_Rotor_M) == 0
      |     fprintf('warning in %s: E_Rotor_M must be a real positive number.\n',gcb)
      | end
      | 
      | % TE_Rotor_Data_M & E_Rotor_Data_M
      | if length(TE_Rotor_Data_M) < 2
      |     fprintf('warning in %s: TE_Rotor_Data_M must have at least 2 elements.\n',gcb)
      | end
      | if length(E_Rotor_Data_M) < 2
      |     fprintf('warning in %s: E_Rotor_Data_M must have at least 2 elements.\n',gcb)
      | end
      | if length(TE_Rotor_Data_M) ~= length(E_Rotor_Data_M)
      |     fprintf('warning in %s: TE_Rotor_Data_M and E_Rotor_Data_M must have the same dimensions.\n',gcb)
      | end
      | real_TE_Rotor_Data_M = isreal(TE_Rotor_Data_M);
      | if min(real_TE_Rotor_Data_M) == 0
      |     fprintf('warning in %s: TE_Rotor_Data_M must have all real entries.\n',gcb)
      | end
      | diff_TE_Rotor_Data_M = diff(TE_Rotor_Data_M);
      | if min(diff_TE_Rotor_Data_M) <= 0
      |     fprintf('warning in %s: TE_Rotor_Data_M must be monotonically increasing.\n',gcb)
      | end
      | if min(TE_Rotor_Data_M) < 0
      |     fprintf('warning in %s: Elements of TE_Rotor_Data_M are below 0 which is theoretically impossible.\n',gcb)
      | end
      | real_E_Rotor_Data_M = isreal(E_Rotor_Data_M);
      | if min(real_E_Rotor_Data_M) == 0
      |     fprintf('warning in %s: E_Rotor_Data_M must have all real entries.\n',gcb)
      | end
      | if min(E_Rotor_Data_M) <= 0
      |     fprintf('warning in %s: Elements of E_Rotor_Data_M are below 0 which is impossible.\n',gcb)
      | end
      | 
      | % v_Rotor_M
      | if length(v_Rotor_M) ~= 1
      |     fprintf('warning in %s: v_Rotor_M must be a scalar entry.\n',gcb)
      | end
      | if isreal(v_Rotor_M) == 0
      |     fprintf('warning in %s: E_Rotor_M must be a real number.\n',gcb)
      | end
      | 
      | % Tv_Rotor_Data_M & v_Rotor_Data_M
      | if length(Tv_Rotor_Data_M) < 2
      |     fprintf('warning in %s: Tv_Rotor_Data_M must have at least 2 elements.\n',gcb)
      | end
      | if length(v_Rotor_Data_M) < 2
      |     fprintf('warning in %s: v_Rotor_Data_M must have at least 2 elements.\n',gcb)
      | end
      | if length(Tv_Rotor_Data_M) ~= length(v_Rotor_Data_M)
      |     fprintf('warning in %s: Tv_Rotor_Data_M and v_Rotor_Data_M must have the same dimensions.\n',gcb)
      | end
      | real_Tv_Rotor_Data_M = isreal(Tv_Rotor_Data_M);
      | if min(real_Tv_Rotor_Data_M) == 0
      |     fprintf('warning in %s: Tv_Rotor_Data_M must have all real entries.\n',gcb)
      | end
      | diff_Tv_Rotor_Data_M = diff(Tv_Rotor_Data_M);
      | if min(diff_Tv_Rotor_Data_M) <= 0
      |     fprintf('warning in %s: Tv_Rotor_Data_M must be monotonically increasing.\n',gcb)
      | end
      | if min(Tv_Rotor_Data_M) < 0
      |     fprintf('warning in %s: Elements of Tv_Rotor_Data_M are below 0 which is theoretically impossible.\n',gcb)
      | end
      | real_E_Rotor_Data_M = isreal(v_Rotor_Data_M);
      | if min(real_E_Rotor_Data_M) == 0
      |     fprintf('warning in %s: v_Rotor_Data_M must have all real entries.\n',gcb)
      | end
      | 
      | % Rotor variables checked by underlying blocks:
      | %   alpha_Rotor_M
      | %   Talpah_Rotor_Data_M
      | %   alpha_Rotor_Data_M
      | 
      | % Case --------------------------%
      | 
      | % W_Case_M
      | if length(W_Case_M) ~= 1
      |     fprintf('warning in %s: W_Case_M must be a scalar entry.\n',gcb)
      | end
      | if W_Case_M <= 0 || isreal(W_Case_M) == 0
      |     fprintf('warning in %s: W_Case_M must be a real positive number.\n',gcb)
      | end
      | 
      | % n_Case_M
      | if length(n_Case_M) ~= 1
      |     fprintf('warning in %s: n_Case_M must be a scalar entry.\n',gcb)
      | end
      | if n_Case_M <= 0 || isreal(n_Case_M) == 0
      |     fprintf('warning in %s: n_Case_M must be a real positive number.\n',gcb)
      | end
      | if n_Case_M < 4
      |     fprintf('warning in %s: n_Case_M must be >= 4.\n',gcb)
      | end
      | 
      | % rho_Case_M
      | if length(rho_Case_M) ~= 1
      |     fprintf('warning in %s: rho_Case_M must be a scalar entry.\n',gcb)
      | end
      | if rho_Case_M <= 0 || isreal(rho_Case_M) == 0
      |     fprintf('warning in %s: rho_Case_M must be a real positive number.\n',gcb)
      | end
      | 
      | % k_Case_M
      | if length(k_Case_M) ~= 1
      |     fprintf('warning in %s: k_Case_M must be a scalar entry.\n',gcb)
      | end
      | if k_Case_M <= 0 || isreal(k_Case_M) == 0
      |     fprintf('warning in %s: k_Case_M must be a real positive number.\n',gcb)
      | end
      | 
      | % Tk_Case_Data_M & k_Case_Data_M
      | if length(Tk_Case_Data_M) < 2
      |     fprintf('warning in %s: Tk_Case_Data_M must have at least 2 elements.\n',gcb)
      | end
      | if length(k_Case_Data_M) < 2
      |     fprintf('warning in %s: k_Case_Data_M must have at least 2 elements.\n',gcb)
      | end
      | if length(Tk_Case_Data_M) ~= length(k_Case_Data_M)
      |     fprintf('warning in %s: Tk_Case_Data_M and k_Case_Data_M must have the same dimensions.\n',gcb)
      | end
      | real_Tk_Case_Data_M = isreal(Tk_Case_Data_M);
      | if min(real_Tk_Case_Data_M) == 0
      |     fprintf('warning in %s: Tk_Case_Data_M must have all real entries.\n',gcb)
      | end
      | diff_Tk_Case_Data_M = diff(Tk_Case_Data_M);
      | if min(diff_Tk_Case_Data_M) <= 0
      |     fprintf('warning in %s: Tk_Case_Data_M must be monotonically increasing.\n',gcb)
      | end
      | if min(Tk_Case_Data_M) < 0
      |     fprintf('warning in %s: Elements of Tk_Case_Data_M are below 0 which is theoretically impossible.\n',gcb)
      | end
      | real_k_Case_Data_M = isreal(k_Case_Data_M);
      | if min(real_k_Case_Data_M) == 0
      |     fprintf('warning in %s: k_Case_Data_M must have all real entries.\n',gcb)
      | end
      | if min(k_Case_Data_M) <= 0
      |     fprintf('warning in %s: Elements of k_Case_Data_M are below 0 which is impossible.\n',gcb)
      | end
      | 
      | % T0_Case_M
      | if length(T0_Case_M) ~= n_Case_M
      |     fprintf('warning in %s: T0_Case_M must be an array with n_Case_M elements.\n',gcb)
      | end
      | real_T0_Case_M = isreal(T0_Case_M);
      | if min(T0_Case_M) <= 0 || min(real_T0_Case_M) == 0
      |     fprintf('warning in %s: T0_Case_M must have all real positive entries.\n',gcb)
      | end
      | 
      | % hcoeff_Case_In_M
      | if length(hcoeff_Case_In_M) ~= 1
      |     fprintf('warning in %s: hcoeff_Case_In_M must be a scalar.\n',gcb)
      | end
      | if hcoeff_Case_In_M < 0 || isreal(hcoeff_Case_In_M) == 0
      |     fprintf('warning in %s: hcoeff_Case_In_M must be a real positive entry.\n',gcb)
      | end
      | 
      | % Wdes_Case_In_M
      | if length(Wdes_Case_In_M) ~= 1
      |     fprintf('warning in %s: Wdes_Case_In_M must be a scalar entry.\n',gcb)
      | end
      | if Wdes_Case_In_M <= 0 || isreal(Wdes_Case_In_M) == 0
      |     fprintf('warning in %s: Wdes_Case_In_M must be a real positive number.\n',gcb)
      | end
      | 
      | % Tdes_Case_In_M
      | if length(Tdes_Case_In_M) ~= 1
      |     fprintf('warning in %s: Tdes_Case_In_M must be a scalar entry.\n',gcb)
      | end
      | if Tdes_Case_In_M <= 0 || isreal(Tdes_Case_In_M) == 0
      |     fprintf('warning in %s: Tdes_Case_In_M must be a real positive number.\n',gcb)
      | end
      | 
      | % Wc_Case_In_Data_M, Tc_Case_In_Data_M & h_Case_In_Data_M
      | [nR, nC] = size(h_Case_In_Data_M);
      | if nR < 2 || nC < 2
      |     fprintf('warning in %s: h_Case_In_Data_M must be a matrix of at least 2 rows and 2 columns.\n',gcb)
      | end
      | if length(Wc_Case_In_Data_M) ~= nR
      |     fprintf('warning in %s: Wc_Case_In_Data_M must have the same number of elements as rows in h_Case_In_Data_M.\n',gcb)
      | end
      | if length(Tc_Case_In_Data_M) ~= nC
      |     fprintf('warning in %s: Tc_Case_In_Data_M must have the same number of elements as columns in h_Case_In_Data_M.\n',gcb)
      | end
      | real_Wc_Case_In_Data_M = isreal(Wc_Case_In_Data_M);
      | if min(real_Wc_Case_In_Data_M) == 0
      |     fprintf('warning in %s: Wc_Case_In_Data_M must have all real entries.\n',gcb)
      | end
      | diff_Wc_Case_In_Data_M = diff(Wc_Case_In_Data_M);
      | if min(diff_Wc_Case_In_Data_M) <= 0
      |     fprintf('warning in %s: Wc_Case_In_Data_M must be monotonically increasing.\n',gcb)
      | end
      | real_Tc_Case_In_Data_M = isreal(Tc_Case_In_Data_M);
      | if min(real_Tc_Case_In_Data_M) == 0
      |     fprintf('warning in %s: Tc_Case_In_Data_M must have all real entries.\n',gcb)
      | end
      | diff_Tc_Case_In_Data_M = diff(Tc_Case_In_Data_M);
      | if min(diff_Tc_Case_In_Data_M) <= 0
      |     fprintf('warning in %s: Tc_Case_In_Data_M must be monotonically increasing.\n',gcb)
      | end
      | if min(Tc_Case_In_Data_M) < 0
      |     fprintf('warning in %s: Elements of Tc_Case_In_Data_M are less than 0 which is impossible.\n',gcb)
      | end
      | real_h_Case_In_Data_M = isreal(h_Case_In_Data_M);
      | if min(real_h_Case_In_Data_M) == 0 || min(min(h_Case_In_Data_M)) < 0
      |     fprintf('warning in %s: h_Case_In_Data_M must have all real positive entries.\n',gcb)
      | end
      | 
      | % hcoeff_Case_Out_M
      | if length(hcoeff_Case_Out_M) ~= 1
      |     fprintf('warning in %s: hcoeff_Case_Out_M must be a scalar.\n',gcb)
      | end
      | if hcoeff_Case_Out_M < 0 || isreal(hcoeff_Case_Out_M) == 0
      |     fprintf('warning in %s: hcoeff_Case_Out_M must be a real positive entry.\n',gcb)
      | end
      | 
      | % Wdes_Case_Out_M
      | if length(Wdes_Case_Out_M) ~= 1
      |     fprintf('warning in %s: Wdes_Case_Out_M must be a scalar entry.\n',gcb)
      | end
      | if Wdes_Case_Out_M <= 0 || isreal(Wdes_Case_Out_M) == 0
      |     fprintf('warning in %s: Wdes_Case_Out_M must be a real positive number.\n',gcb)
      | end
      | 
      | % Tdes_Case_Out_M
      | if length(Tdes_Case_Out_M) ~= 1
      |     fprintf('warning in %s: Tdes_Case_Out_M must be a scalar entry.\n',gcb)
      | end
      | if Tdes_Case_Out_M <= 0 || isreal(Tdes_Case_Out_M) == 0
      |     fprintf('warning in %s: Tdes_Case_Out_M must be a real positive number.\n',gcb)
      | end
      | 
      | % Wc_Case_Out_Data_M, Tc_Case_Out_Data_M & h_Case_Out_Data_M
      | [nR, nC] = size(h_Case_Out_Data_M);
      | if nR < 2 || nC < 2
      |     fprintf('warning in %s: h_Case_Out_Data_M must be a matrix of at least 2 rows and 2 columns.\n',gcb)
      | end
      | if length(Wc_Case_Out_Data_M) ~= nR
      |     fprintf('warning in %s: Wc_Case_Out_Data_M must have the same number of elements as rows in h_Case_Out_Data_M.\n',gcb)
      | end
      | if length(Tc_Case_Out_Data_M) ~= nC
      |     fprintf('warning in %s: Tc_Case_Out_Data_M must have the same number of elements as columns in h_Case_Out_Data_M.\n',gcb)
      | end
      | real_Wc_Case_Out_Data_M = isreal(Wc_Case_Out_Data_M);
      | if min(real_Wc_Case_Out_Data_M) == 0
      |     fprintf('warning in %s: Wc_Case_Out_Data_M must have all real entries.\n',gcb)
      | end
      | diff_Wc_Case_Out_Data_M = diff(Wc_Case_Out_Data_M);
      | if min(diff_Wc_Case_Out_Data_M) <= 0
      |     fprintf('warning in %s: Wc_Case_Out_Data_M must be monotonically increasing.\n',gcb)
      | end
      | real_Tc_Case_Out_Data_M = isreal(Tc_Case_Out_Data_M);
      | if min(real_Tc_Case_Out_Data_M) == 0
      |     fprintf('warning in %s: Tc_Case_Out_Data_M must have all real entries.\n',gcb)
      | end
      | diff_Tc_Case_Out_Data_M = diff(Tc_Case_Out_Data_M);
      | if min(diff_Tc_Case_Out_Data_M) <= 0
      |     fprintf('warning in %s: Tc_Case_Out_Data_M must be monotonically increasing.\n',gcb)
      | end
      | if min(Tc_Case_Out_Data_M) < 0
      |     fprintf('warning in %s: Elements of Tc_Case_Out_Data_M are less than 0 which is impossible.\n',gcb)
      | end
      | real_h_Case_Out_Data_M = isreal(h_Case_Out_Data_M);
      | if min(real_h_Case_Out_Data_M) == 0 || min(min(h_Case_Out_Data_M)) < 0
      |     fprintf('warning in %s: h_Case_Out_Data_M must have all real positive entries.\n',gcb)
      | end
      | 
      | % Ri_Case_M
      | if length(Ri_Case_M) ~= 1
      |     fprintf('warning in %s: Ri_Case_M must be a scalar entry.\n',gcb)
      | end
      | if Ri_Case_M <= 0 || isreal(Ri_Case_M) == 0
      |     fprintf('warning in %s: Ri_Case_M must be a real positive number.\n',gcb)
      | end
      | 
      | % L_Shroud_M
      | if length(L_Shroud_M) ~= 1
      |     fprintf('warning in %s: L_Shroud_M must be a scalar entry.\n',gcb)
      | end
      | if L_Shroud_M <= 0 || isreal(L_Shroud_M) == 0
      |     fprintf('warning in %s: L_Shroud_M must be a real positive number.\n',gcb)
      | end
      | 
      | % Case variables checked by underlying blocks:
      | %   alpha_Case_M
      | %   Talpha_Case_Data_M
      | %   alpha_Case_data_M
      | 
      | % calculate intialization parameters -------------------------------------%
      | 
      | % Rotor discretization (node locations)
      | dx_Rotor = W_Rotor_M/(n_Rotor_M-0.5); %node thickness
      | x_Rotor_I = [0:dx_Rotor:W_Rotor_M]; %discretization array [ft]
      | 
      | % Case discretization (nodel locations)
      | dx_Case = W_Case_M/(n_Case_M-1); %node thickness
      | x_Case_I = Ri_Case_M + [0:dx_Case:W_Case_M]; %discretizaiton array [ft]
      | 
      | % Convection Model selection variables
      | % Blade
      | if h_Const_Blade_M == 1
      |     ConvHeatXCoeffMdl_Blade_I = 1;
      | elseif h_Eqn_Blade_M == 1
      |     ConvHeatXCoeffMdl_Blade_I = 2;
      | elseif h_Data_Blade_M == 1
      |     ConvHeatXCoeffMdl_Blade_I = 3;
      | end
      | % Rotor-Front
      | if h_Const_Rotor_Front_M == 1
      |     ConvHeatXCoeffMdl_Rotor_Front_I = 1;
      | elseif h_Eqn_Rotor_Front_M == 1
      |     ConvHeatXCoeffMdl_Rotor_Front_I = 2;
      | elseif h_Data_Rotor_Front_M == 1
      |     ConvHeatXCoeffMdl_Rotor_Front_I = 3;
      | end
      | % Rotor-Back
      | if h_Const_Rotor_Back_M == 1
      |     ConvHeatXCoeffMdl_Rotor_Back_I = 1;
      | elseif h_Eqn_Rotor_Back_M == 1
      |     ConvHeatXCoeffMdl_Rotor_Back_I = 2;
      | elseif h_Data_Rotor_Back_M == 1
      |     ConvHeatXCoeffMdl_Rotor_Back_I = 3;
      | end
      | % Case-In
      | if h_Const_Case_In_M == 1
      |     ConvHeatXCoeffMdl_Case_In_I = 1;
      | elseif h_Eqn_Case_In_M == 1
      |     ConvHeatXCoeffMdl_Case_In_I = 2;
      | elseif h_Data_Case_In_M == 1
      |     ConvHeatXCoeffMdl_Case_In_I = 3;
      | end
      | % Case-Out
      | if h_Const_Case_Out_M == 1
      |     ConvHeatXCoeffMdl_Case_Out_I = 1;
      | elseif h_Eqn_Case_Out_M == 1
      |     ConvHeatXCoeffMdl_Case_Out_I = 2;
      | elseif h_Data_Case_Out_M == 1
      |     ConvHeatXCoeffMdl_Case_Out_I = 3;
      | end
      | 
      | % set thermal expansion temperature dependence settings ------------------%
      | 
      | % Blade
      | set_param([gcb,'/Blade Deformation/Deformation/Deformation Due To Thermal Expansion/Thermal Expansion 1D Elastic'],'TempDependence_M',alpha_TempDependence_Blade_M);
      |     
      | % Rotor
      | set_param([gcb,'/Rotor Deformation/Deformation/Deformation Due To Thermal Expansion/Thermal Expansion 1D Elastic'],'TempDependence_M',alpha_TempDependence_Rotor_M);
      | 
      | % Case
      | set_param([gcb,'/Case Deformation/Deformation/Thermal Expansion 1D Elastic'],'TempDependence_M',alpha_TempDependence_Case_M);
      | 
      | % set default parameters if they are not being used ----------------------%
      | 
      | % Blade
      | if h_Const_Blade_M == 1
      |     hcoeff_Blade_M = 0.003;
      |     Wdes_Blade_M = 1;
      |     Tdes_Blade_M = 1;
      |     Wc_Blade_Data_M = [0 10000];
      |     Tc_Blade_Data_M = [0 10000];
      |     h_Blade_Data_M = [0.003 0.003; 0.003 0.003];
      | elseif h_Eqn_Blade_M == 1
      |     h_Blade_M = 0.003;
      |     Wc_Blade_Data_M = [0 10000];
      |     Tc_Blade_Data_M = [0 10000];
      |     h_Blade_Data_M = [0.003 0.003; 0.003 0.003];
      | elseif h_Data_Blade_M == 1
      |     h_Blade_M = 0.003;
      |     hcoeff_Blade_M = 0.003;
      | end
      | 
      | if alpha_TempDependence_Blade_M == 0
      |     Talpha_Blade_Data_M = [0 10000];
      |     alpha_Blade_Data_M = [0.000001 0.000001];
      | elseif alpha_TempDependence_Blade_M == 1
      |     alpha_Blade_M = 0.000001;
      | end
      | 
      | if E_TempDependence_Blade_M == 0
      |     TE_Blade_Data_M = [0 10000];
      |     E_Blade_Data_M = [3974400000 3974400000];
      | elseif E_TempDependence_Blade_M == 1
      |     E_Blade_M = 3974400000;
      | end
      | 
      | % Rotor
      | if k_TempDependence_Rotor_M == 0
      |     Tk_Rotor_Data_M = [0 10000];
      |     k_Rotor_Data_M = [0.0015 0.0015];
      | elseif k_TempDependence_Rotor_M == 1
      |     k_Rotor_M = 0.0015;
      | end
      | 
      | if h_Const_Rotor_Front_M == 1
      |     hcoeff_Rotor_Front_M = 0.003;
      |     Wdes_Rotor_Front_M = 1;
      |     Tdes_Rotor_Front_M = 1;
      |     Wc_Rotor_Front_Data_M = [0 10000];
      |     Tc_Rotor_Front_Data_M = [0 10000];
      |     h_Rotor_Front_Data_M = [0.003 0.003; 0.003 0.003];
      | elseif h_Eqn_Rotor_Front_M == 1
      |     h_Rotor_Front_M = 0.003;
      |     Wc_Rotor_Front_Data_M = [0 10000];
      |     Tc_Rotor_Front_Data_M = [0 10000];
      |     h_Rotor_Front_Data_M = [0.003 0.003; 0.003 0.003];
      | elseif h_Data_Rotor_Front_M == 1
      |     h_Rotor_Front_M = 0.003;
      |     hcoeff_Rotor_Front_M = 0.003;
      | end
      | 
      | if h_Const_Rotor_Back_M == 1
      |     hcoeff_Rotor_Back_M = 0.003;
      |     Wdes_Rotor_Back_M = 1;
      |     Tdes_Rotor_Back_M = 1;
      |     Wc_Rotor_Back_Data_M = [0 10000];
      |     Tc_Rotor_Back_Data_M = [0 10000];
      |     h_Rotor_Back_Data_M = [0.003 0.003; 0.003 0.003];
      | elseif h_Eqn_Rotor_Back_M == 1
      |     h_Rotor_Back_M = 0.003;
      |     Wc_Rotor_Back_Data_M = [0 10000];
      |     Tc_Rotor_Back_Data_M = [0 10000];
      |     h_Rotor_Back_Data_M = [0.003 0.003; 0.003 0.003];
      | elseif h_Data_Rotor_Back_M == 1
      |     h_Rotor_Back_M = 0.003;
      |     hcoeff_Rotor_Back_M = 0.003;
      | end
      | 
      | if alpha_TempDependence_Rotor_M == 0
      |     Talpha_Rotor_Data_M = [0 10000];
      |     alpha_Rotor_Data_M = [0.000001 0.000001];
      | elseif alpha_TempDependence_Rotor_M == 1
      |     alpha_Rotor_M = 0.000001;
      | end
      | 
      | if E_TempDependence_Rotor_M == 0
      |     TE_Rotor_Data_M = [0 10000];
      |     E_Rotor_Data_M = [3974400000 3974400000];
      | elseif E_TempDependence_Rotor_M == 1
      |     E_Rotor_M = 3974400000;
      | end
      | 
      | if v_TempDependence_Rotor_M == 0
      |     Tv_Rotor_Data_M = [0 10000];
      |     v_Rotor_Data_M = [0.3 0.3];
      | elseif v_TempDependence_Rotor_M == 1
      |     v_Rotor_M = 0.3;
      | end
      | 
      | % Case
      | if k_TempDependence_Case_M == 0
      |     Tk_Case_Data_M = [0 10000];
      |     k_Case_Data_M = [0.0015 0.0015];
      | elseif k_TempDependence_Case_M == 1
      |     k_Case_M = 0.0015;
      | end
      | 
      | if h_Const_Case_In_M == 1
      |     hcoeff_Case_In_M = 0.003;
      |     Wdes_Case_In_M = 1;
      |     Tdes_Case_In_M = 1;
      |     Wc_Case_In_Data_M = [0 10000];
      |     Tc_Case_In_Data_M = [0 10000];
      |     h_Case_In_Data_M = [0.003 0.003; 0.003 0.003];
      | elseif h_Eqn_Case_In_M == 1
      |     h_Case_In_M = 0.003;
      |     Wc_Case_In_Data_M = [0 10000];
      |     Tc_Case_In_Data_M = [0 10000];
      |     h_Case_In_Data_M = [0.003 0.003; 0.003 0.003];
      | elseif h_Data_Case_In_M == 1
      |     h_Case_In_M = 0.003;
      |     hcoeff_Case_In_M = 0.003;
      | end
      | 
      | if h_Const_Case_Out_M == 1
      |     hcoeff_Case_Out_M = 0.003;
      |     Wdes_Case_Out_M = 1;
      |     Tdes_Case_Out_M = 1;
      |     Wc_Case_Out_Data_M = [0 10000];
      |     Tc_Case_Out_Data_M = [0 10000];
      |     h_Case_Out_Data_M = [0.003 0.003; 0.003 0.003];
      | elseif h_Eqn_Case_Out_M == 1
      |     h_Case_Out_M = 0.003;
      |     Wc_Case_Out_Data_M = [0 10000];
      |     Tc_Case_Out_Data_M = [0 10000];
      |     h_Case_Out_Data_M = [0.003 0.003; 0.003 0.003];
      | elseif h_Data_Case_Out_M == 1
      |     h_Case_Out_M = 0.003;
      |     hcoeff_Case_Out_M = 0.003;
      | end
      | 
      | if alpha_TempDependence_Case_M == 0
      |     Talpha_Case_Data_M = [0 10000];
      |     alpha_Case_Data_M = [0.000001 0.000001];
      | elseif alpha_TempDependence_Case_M == 1
      |     alpha_Case_M = 0.000001;
      | end
      | 
      | % inport and constant block swapping -------------------------------------%
      | 
      | % Inport Numbers
      | n = 4; %first inport number
      | 
      | % Rotor Cooling Flow Mass Flow Rate - Front Inport
      | n = n + 1;
      | if h_Const_Rotor_Front_M == 0
      |     if strcmp(get_param([gcb '/Wcool - Rotor Front (slug//sec)'],'BlockType'),'Constant')
      |         MSK_ReplaceBlock_TMATS([gcb '/Wcool - Rotor Front (slug//sec)'],'built-in/Inport');
      |     end
      |     set_param([gcb '/Wcool - Rotor Front (slug//sec)'],'Port',num2str(n));
      |     n = n + 1;
      | else
      |     if strcmp(get_param([gcb '/Wcool - Rotor Front (slug//sec)'],'BlockType'),'Inport')
      |         MSK_ReplaceBlock_TMATS([gcb '/Wcool - Rotor Front (slug//sec)'],'built-in/Constant');
      |         set_param([gcb '/Wcool - Rotor Front (slug//sec)'],'Value','1');
      |     end
      | end
      | 
      | % Rotor Cooling Flow Mass Flow Rate - Back Inport
      | n = n + 1;
      | if h_Const_Rotor_Back_M == 0
      |     if strcmp(get_param([gcb '/Wcool - Rotor Back (slug//sec)'],'BlockType'),'Constant')
      |         MSK_ReplaceBlock_TMATS([gcb '/Wcool - Rotor Back (slug//sec)'],'built-in/Inport');
      |     end
      |     set_param([gcb '/Wcool - Rotor Back (slug//sec)'],'Port',num2str(n));
      |     n = n + 1;
      | else
      |     if strcmp(get_param([gcb '/Wcool - Rotor Back (slug//sec)'],'BlockType'),'Inport')
      |         MSK_ReplaceBlock_TMATS([gcb '/Wcool - Rotor Back (slug//sec)'],'built-in/Constant');
      |         set_param([gcb '/Wcool - Rotor Back (slug//sec)'],'Value','1');
      |     end
      | end
      | 
      | % Case Cooling Flow Mass Flow Rate - Inner Inport
      | n = n + 1;
      | if h_Const_Case_In_M == 0
      |     if strcmp(get_param([gcb '/Win - Case (slug//sec)'],'BlockType'),'Constant')
      |         MSK_ReplaceBlock_TMATS([gcb '/Win - Case (slug//sec)'],'built-in/Inport');
      |     end
      |     set_param([gcb '/Win - Case (slug//sec)'],'Port',num2str(n));
      |     n = n + 1;
      | else
      |     if strcmp(get_param([gcb '/Win - Case (slug//sec)'],'BlockType'),'Inport')
      |         MSK_ReplaceBlock_TMATS([gcb '/Win - Case (slug//sec)'],'built-in/Constant');
      |         set_param([gcb '/Win - Case (slug//sec)'],'Value','1');
      |     end
      | end
      | 
      | % Case Cooling Flow Mass Flow Rate - Outer Inport
      | n = n + 1;
      | if h_Const_Case_Out_M == 0
      |     if strcmp(get_param([gcb '/Wout - Case (slug//sec)'],'BlockType'),'Constant')
      |         MSK_ReplaceBlock_TMATS([gcb '/Wout - Case (slug//sec)'],'built-in/Inport');
      |     end
      |     set_param([gcb '/Wout - Case (slug//sec)'],'Port',num2str(n));
      |     n = n + 1;
      | else
      |     if strcmp(get_param([gcb '/Wout - Case (slug//sec)'],'BlockType'),'Inport')
      |         MSK_ReplaceBlock_TMATS([gcb '/Wout - Case (slug//sec)'],'built-in/Constant');
      |         set_param([gcb '/Wout - Case (slug//sec)'],'Value','1');
      |     end
      | end
      mask Help: web(which('SSTipClearance.html'),'-helpbrowser')
      mask Callback h_Const_Blade_M:
      | if length(get_param(gcb,'h_Const_Blade_M')) == 2 %on
      |     set_param(gcb,'h_Eqn_Blade_M','off');
      |     set_param(gcb,'h_Data_Blade_M','off');
      |     MSK_SEC_Enables2_TMATS('h_Const_Blade_M',6,'en')
      |     MSK_SEC_Enables2_TMATS('h_Const_Blade_M',[7 8 9 10 11 12],'dis')
      | end
      mask Callback h_Eqn_Blade_M:
      | if length(get_param(gcb,'h_Eqn_Blade_M')) == 2 %on
      |     set_param(gcb,'h_Const_Blade_M','off');
      |     set_param(gcb,'h_Data_Blade_M','off');
      |     MSK_SEC_Enables2_TMATS('h_Eqn_Blade_M',[7 8 9],'en')
      |     MSK_SEC_Enables2_TMATS('h_Eqn_Blade_M',[6 10 11 12],'dis')
      | end
      mask Callback h_Data_Blade_M:
      | if length(get_param(gcb,'h_Data_Blade_M')) == 2 %on
      |     set_param(gcb,'h_Eqn_Blade_M','off');
      |     set_param(gcb,'h_Const_Blade_M','off');
      |     MSK_SEC_Enables2_TMATS('h_Data_Blade_M',[6 7],'dis')
      |     MSK_SEC_Enables2_TMATS('h_Data_Blade_M',[8 9 10 11 12],'en')
      | end
      mask Callback alpha_TempDependence_Blade_M:
      | MSK_SEC_Enables_TMATS('alpha_TempDependence_Blade_M',16,'dis')
      | MSK_SEC_Enables_TMATS('alpha_TempDependence_Blade_M',[17 18],'en')
      mask Callback E_TempDependence_Blade_M:
      | MSK_SEC_Enables_TMATS('E_TempDependence_Blade_M',20,'dis')
      | MSK_SEC_Enables_TMATS('E_TempDependence_Blade_M',[21 22],'en')
      mask Callback k_TempDependence_Rotor_M:
      | MSK_SEC_Enables_TMATS('k_TempDependence_Rotor_M',28,'dis')
      | MSK_SEC_Enables_TMATS('k_TempDependence_Rotor_M',[29 30],'en')
      mask Callback h_Const_Rotor_Front_M:
      | if length(get_param(gcb,'h_Const_Rotor_Front_M')) == 2 %on
      |     set_param(gcb,'h_Eqn_Rotor_Front_M','off');
      |     set_param(gcb,'h_Data_Rotor_Front_M','off');
      |     MSK_SEC_Enables2_TMATS('h_Const_Rotor_Front_M',34,'en')
      |     MSK_SEC_Enables2_TMATS('h_Const_Rotor_Front_M',[35 36 37 38 39 40],'dis')
      | end
      mask Callback h_Eqn_Rotor_Front_M:
      | if length(get_param(gcb,'h_Eqn_Rotor_Front_M')) == 2 %on
      |     set_param(gcb,'h_Const_Rotor_Front_M','off');
      |     set_param(gcb,'h_Data_Rotor_Front_M','off');
      |     MSK_SEC_Enables2_TMATS('h_Eqn_Rotor_Front_M',[35 36 37],'en')
      |     MSK_SEC_Enables2_TMATS('h_Eqn_Rotor_Front_M',[34 38 39 40],'dis')
      | end
      mask Callback h_Data_Rotor_Front_M:
      | if length(get_param(gcb,'h_Data_Rotor_Front_M')) == 2 %on
      |     set_param(gcb,'h_Eqn_Rotor_Front_M','off');
      |     set_param(gcb,'h_Const_Rotor_Front_M','off');
      |     MSK_SEC_Enables2_TMATS('h_Data_Rotor_Front_M',[34 35],'dis')
      |     MSK_SEC_Enables2_TMATS('h_Data_Rotor_Front_M',[36 37 38 39 40],'en')
      | end
      mask Callback h_Const_Rotor_Back_M:
      | if length(get_param(gcb,'h_Const_Rotor_Back_M')) == 2 %on
      |     set_param(gcb,'h_Eqn_Rotor_Back_M','off');
      |     set_param(gcb,'h_Data_Rotor_Back_M','off');
      |     MSK_SEC_Enables2_TMATS('h_Const_Rotor_Back_M',44,'en')
      |     MSK_SEC_Enables2_TMATS('h_Const_Rotor_Back_M',[45 46 47 48 49 50],'dis')
      | end
      mask Callback h_Eqn_Rotor_Back_M:
      | if length(get_param(gcb,'h_Eqn_Rotor_Back_M')) == 2 %on
      |     set_param(gcb,'h_Const_Rotor_Back_M','off');
      |     set_param(gcb,'h_Data_Rotor_Back_M','off');
      |     MSK_SEC_Enables2_TMATS('h_Eqn_Rotor_Back_M',[45 46 47],'en')
      |     MSK_SEC_Enables2_TMATS('h_Eqn_Rotor_Back_M',[44 48 49 50],'dis')
      | end
      mask Callback h_Data_Rotor_Back_M:
      | if length(get_param(gcb,'h_Data_Rotor_Back_M')) == 2 %on
      |     set_param(gcb,'h_Eqn_Rotor_Back_M','off');
      |     set_param(gcb,'h_Const_Rotor_Back_M','off');
      |     MSK_SEC_Enables2_TMATS('h_Data_Rotor_Back_M',[44 45],'dis')
      |     MSK_SEC_Enables2_TMATS('h_Data_Rotor_Back_M',[46 47 48 49 50],'en')
      | end
      mask Callback alpha_TempDependence_Rotor_M:
      | MSK_SEC_Enables_TMATS('alpha_TempDependence_Rotor_M',53,'dis')
      | MSK_SEC_Enables_TMATS('alpha_TempDependence_Rotor_M',[54 55],'en')
      mask Callback E_TempDependence_Rotor_M:
      | MSK_SEC_Enables_TMATS('E_TempDependence_Rotor_M',57,'dis')
